simulink library "MCHP_Blockset"  (R2014b)
settings: Solver=ode45  SolverMode=SingleTasking  StartTime=0.0  StopTime=10.0  RelTol=1e-3
InitFcn:
  | disp('MCHP_Blockset_Library_InitFunction');
undefined symbols (not defined in the file): A0, A2, AD0, AVdd, B1, B5, B9, C10, C2, CMP2A, CMP3A, CMP4A, EXTREF1, EXTREF2, gcbh, MaxPer, MCHP_ACC_SAMx_Callback, MCHP_ADC_Callback, MCHP_ADC_HighSpeed_SAR_Callback, MCHP_ADC_HighSpeed_SAR_dsPIC_Callback, MCHP_ADC_SAME5x_Callback, MCHP_AFEC_SAM7x_Callback, MCHP_BUS_I2C_MASTER_callback, MCHP_BUS_SPI_callback, MCHP_C_function_Call_callback, MCHP_CN_Callback, MCHP_COMPARATOR1_callback, MCHP_CompilerOptimisation_Callback, MCHP_DACC_SAMx_Callback, MCHP_Digital_Input_Callback, MCHP_Digital_Output_Read_Callback, MCHP_Digital_Output_Write_Callback, MCHP_Fun, MCHP_HighSpeed_AnalogComparator_Callback, MCHP_IC_Callback, MCHP_IdleTask_Callback, MCHP_Interrupt_Callback, MCHP_Master_Callback, MCHP_MCPWM_Callback, MCHP_MCU_LOAD_Callback, MCHP_MCU_OVERLOAD_Callback, MCHP_MSI_Callback, MCHP_OC_HW_Callback, MCHP_OC_SW_Callback, MCHP_OP_AMP_Callback, MCHP_OrderInOut, MCHP_PDEC_Callback, MCHP_PGA_Callback, MCHP_PWM_Callback, MCHP_PWM_HighSpeed_Override_Callback, MCHP_PWM_HS_FEP_Callback, MCHP_PWM_SAM7x_Callback, MCHP_PWM_SAM7x_Override_Callback, MCHP_QDEC_SAMx_Callback, MCHP_QEI_Callback, MCHP_Scheduler_Options_Callback, MCHP_SECONDARY_CORE_Callback, MCHP_Tasks_State_Callback, MCHP_TCC_PWM_Callback, MCHP_TIMER_Config_Callback ... (+18)
libraries: MCHP_Blockset x2
(part 5 of 9)

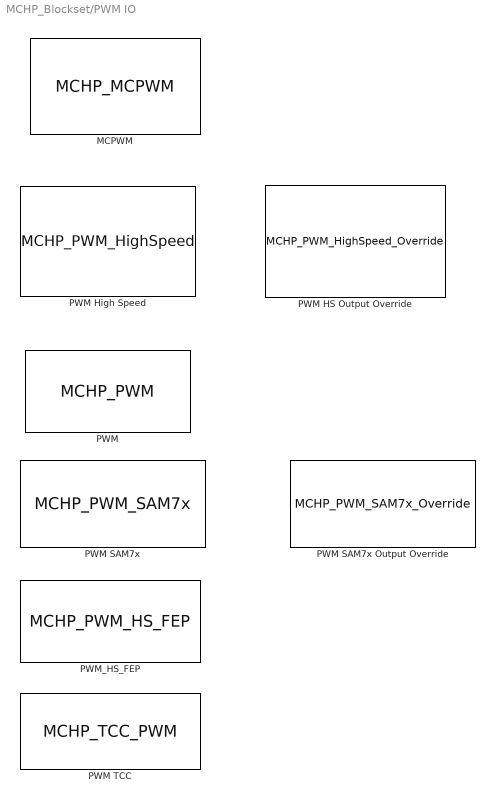
== system MCHP_Blockset/PWM IO ==
  MCPWM : S-Function  Priority=-2000  LoadFcn=MCHP_Fun.Load_EvalIn_ws(gcbh);  InitFcn=MCHP_MCPWM_Callback(gcbh,'InitFcn');  FunctionName=MCHP_MCPWM  Parameters=MCHP_MCPWM_Callback(gcbh,'S_INPUT'),MCHP_MCPWM_Callback(gcbh,'S_OUTPUT'),MCHP_MCPWM_Callback(gcbh,'S_INPUT_Size'),MCHP_MCPWM_Callback(gcbh,'S_OUTPUT_Size'),MCHP_MCPWM_Callback(gcbh,'S_ListCustomDatatype'),SampleTime,0  EnableBusSupport=off  mask(MCPWM PIC32 EF family){PWMx_ECAM_ITB=Common - Edge aligned, PWMx_MTBS=Primary master timer, PWM_ClockResolution=Dynamic Options, PWM_ClockResolution_TXT=auto, MaxPeriod_s=50e-6, InitPeriode_s=50e-6, InitDutyCycleP_s=20e-6, InitDutyCycleS_s=10e-6, InitPhase_s=-1, SampleTime=-1, S_INPUT=[-1], S_INPUT_Size=[3], S_OUTPUT=[], S_OUTPUT_Size=[], S_ListCustomDatatype=S.S_ListCustomDatatype={};, MCHP_USER_INTERRUPTS=0, evalin_ws='', MCHP_PORT={PWMH1 }{PWMH1}32:4:B14;{PWMH2 }{PWMH2}32:4:B12;{PWMH3 }{PWMH3}32:4:B10;{PWML1}{PWML1}32:4:B15;{PWML2}{PWML2}32:4:B13;{PWML3}{PWML3}32:4:B11;, MCHP_MASTERLINK=Export_To_Lib/Microchip Master, MCHP_CRC=1635607, INFO=, PWMx_PMOD=Complementary, PWM1_HL=PWMxH & PWMxL output enabled, PWM1_swap=off, PWM1H_pol=off, PWM1L_pol=off, PWM2_HL=PWMxH & PWMxL output enabled, PWM2_swap=off, PWM2H_pol=off, PWM2L_pol=off, PWM3_HL=PWMxH & PWMxL output enabled, PWM3_swap=off, PWM3H_pol=off, PWM3L_pol=off, PWM4_HL=not used, PWM4_swap=off, PWM4H_pol=off, PWM4L_pol=off, PWM5_HL=not used, PWM5_swap=off, PWM5H_pol=off, PWM5L_pol=off, PWM6_HL=not used, PWM6_swap=off, PWM6H_pol=off, PWM6L_pol=off, PWM7_HL=not used, PWM7_swap=off, PWM7H_pol=off, PWM7L_pol=off, PWM8_HL=not used, PWM8_swap=off, PWM8H_pol=off, PWM8L_pol=off, PWM9_HL=not used, PWM9_swap=off, PWM9H_pol=off, PWM9L_pol=off, PWM10_HL=not used, PWM10_swap=off, PWM10H_pol=off, PWM10L_pol=off, PWM11_HL=not used, PWM11_swap=off, PWM11H_pol=off, PWM11L_pol=off, PWM12_HL=not used, PWM12_swap=off, PWM12H_pol=off, PWM12L_pol=off, Init_SEVTCMP_SSEVTCMP=-1, Init_TRIGx_STRIGx_1=[-1 -1], Init_TRIGx_STRIGx_2=[-1 -1], Init_TRIGx_STRIGx_3=[-1 -1], Init_TRIGx_STRIGx_4=[-1 -1], Init_TRIGx_STRIGx_5=[-1 -1], Init_TRIGx_STRIGx_6=[-1 -1], Init_TRIGx_STRIGx_7=[-1 -1], Init_TRIGx_STRIGx_8=[-1 -1], Init_TRIGx_STRIGx_9=[-1 -1], Init_TRIGx_STRIGx_10=[-1 -1], Init_TRIGx_STRIGx_11=[-1 -1], Init_TRIGx_STRIGx_12=[-1 -1], TRIG_DualTriggerMode=Primary Trigger to ADC is independant, BlockInput_VectorScalar=Vectors (grouped by function), BlockInput_Period=Not a block input, BlockInput_DutyCycle=a Floating Point input within range [0 1], BlockInput_PhaseShift=Not a block input, BlockInput_SEVTCMP=Not a block input, BlockInput_TRIGx=Not a block input, BlockInput_DeadTime=Not a block input, BlockOutput_FaultDisabled=off, BlockOutput_Fault=on, DTC=Disabled, FLTSRC1_DTCMP=Dynamic Options, FLTSRC1_DTCMP_TXT=FLT6 / E13 / Pin[42]  -  Active HIGH, FLTSRC2_DTCMP=Dynamic Options, FLTSRC2_DTCMP_TXT=FLT6 / E13 / Pin[42]  -  Active LOW, FLTSRC3_DTCMP=Dynamic Options, FLTSRC3_DTCMP_TXT=FLT8 / E15 / Pin[44]  -  Active LOW, FLTSRC4_DTCMP=Dynamic Options, FLTSRC4_DTCMP_TXT=FLT3 / C2 / Pin[34]  -  Active HIGH, FLTSRC5_DTCMP=Dynamic Options, FLTSRC5_DTCMP_TXT=FLT3 / C2 / Pin[34]  -  Active HIGH, FLTSRC6_DTCMP=Dynamic Options, FLTSRC6_DTCMP_TXT=FLT3 / C2 / Pin[34]  -  Active HIGH, FLTSRC7_DTCMP=Dynamic Options, FLTSRC7_DTCMP_TXT=FLT3 / C2 / Pin[34]  -  Active HIGH, FLTSRC8_DTCMP=Dynamic Options, FLTSRC8_DTCMP_TXT=FLT3 / C2 / Pin[34]  -  Active HIGH, FLTSRC9_DTCMP=Dynamic Options, FLTSRC9_DTCMP_TXT=FLT3 / C2 / Pin[34]  -  Active HIGH, FLTSRC10_DTCMP=Dynamic Options, FLTSRC10_DTCMP_TXT=FLT3 / C2 / Pin[34]  -  Active HIGH, FLTSRC11_DTCMP=Dynamic Options, FLTSRC11_DTCMP_TXT=FLT3 / C2 / Pin[34]  -  Active HIGH, FLTSRC12_DTCMP=Dynamic Options, FLTSRC12_DTCMP_TXT=FLT3 / C2 / Pin[34]  -  Active HIGH, DeadTime_s=2e-6, DeadTimeAlt_s=2e-6, DeadTimeComp_s=0, FLTMODx=Disabled, FLTSRCx=Dynamic Options, FLTSRCx_TXT=FLT3 / C2 / Pin[34]  -  Active HIGH, FLTDATx=PWM H/L -> 11, CLMODx=Disabled, CLSRCx=Dynamic Options, CLSRCx_TXT=FLT8 / E15 / Pin[44]  -  Active LOW, CLDATx=PWM H/L -> 00, FLTLEBENx=off, CLLEBENx=off, LeadEdgeBlkPer_s=5e-7, PHRx=off, PHFx=off, PLRx=off, PLFx=off}
      mask prompts: PWMx_ECAM_ITB "Period :"; PWMx_MTBS "Clock source :"; PWM_ClockResolution "Clock source resolution : [PWM res 8.333(ns) => periode up to 546(us) ]"; PWM_ClockResolution_TXT "<empty>"; MaxPeriod_s "Max Period (s) : PWM1max=PWM2max=PWM3max=6000 (12.55bits width)  represent 50(us)"; InitPeriode_s "Initial Period (s) :"; InitDutyCycleP_s "Initial Duty Cycle (s)"; InitDutyCycleS_s "Initial second half Duty Cycle (s)"; InitPhase_s "Initial Phase (s) :"; SampleTime "Block output sample time"; INFO "Infos"; PWMx_PMOD "High/Low side Mode :"; PWM1_HL "PWM 1 Channel"; PWM1_swap "Swap PWM1_H and PWM1_L"; PWM1H_pol "invert PWM1_H output polarity ( B14 [4] active low )"; PWM1L_pol "invert PWM1_L output polarity ( B15 [5] active low )"; PWM2_HL "PWM 2 Channel"; PWM2_swap "Swap PWM2_H and PWM2_L"; PWM2H_pol "invert PWM2_H output polarity ( B12 [98] active low )"; PWM2L_pol "invert PWM2_L output polarity ( B13 [99] active low )"; PWM3_HL "PWM 3 Channel"; PWM3_swap "Swap PWM3_H and PWM3_L"; PWM3H_pol "invert PWM3_H output polarity ( B10 [93] active low )"; PWM3L_pol "invert PWM3_L output polarity ( B11 [94] active low )"; PWM4_HL "PWM 4 Channel"; PWM4_swap "Swap PWM4_H and PWM4_L"; PWM4H_pol "invert PWM4_H output polarity ( A10 [100] active low )"; PWM4L_pol "invert PWM4_L output polarity ( A7 [3] active low )"; PWM5_HL "PWM 5 Channel"; PWM5_swap "Swap PWM5_H and PWM5_L"; PWM5H_pol "invert PWM5_H output polarity ( D2 [7] active low )"; PWM5L_pol "invert PWM5_L output polarity ( D1 [6] active low )"; PWM6_HL "PWM 6 Channel"; PWM6_swap "Swap PWM6_H and PWM6_L"; PWM6H_pol "invert PWM6_H output polarity ( D4 [9] active low )"; PWM6L_pol "invert PWM6_L output polarity ( D3 [8] active low )"; PWM7_HL "PWM 7 Channel"; PWM7_swap "Swap PWM7_H and PWM7_L"; PWM7H_pol "invert PWM7_H output polarity ( B15 [5] active low )"; PWM7L_pol "<empty>"; PWM8_HL "PWM 8 Channel"; PWM8_swap "Swap PWM8_H and PWM8_L"; PWM8H_pol "invert PWM8_H output polarity ( B13 [99] active low )"; PWM8L_pol "<empty>"; PWM9_HL "PWM 9 Channel"; PWM9_swap "Swap PWM9_H and PWM9_L"; PWM9H_pol "invert PWM9_H output polarity ( B11 [94] active low )"; PWM9L_pol "<empty>"; PWM10_HL "PWM 10 Channel"; PWM10_swap "Swap PWM10_H and PWM10_L"; PWM10H_pol "invert PWM10_H output polarity ( A7 [3] active low )"; PWM10L_pol "<empty>"; PWM11_HL "PWM 11 Channel"; PWM11_swap "Swap PWM11_H and PWM11_L"; PWM11H_pol "invert PWM11_H output polarity ( F0 [87] active low )"; PWM11L_pol "invert PWM11_L output polarity ( F1 [88] active low )"; PWM12_HL "PWM 12 Channel"; PWM12_swap "Swap PWM12_H and PWM12_L"; PWM12H_pol "invert PWM12_H output polarity ( D5 [82] active low )"; PWM12L_pol "invert PWM12_L output polarity ( D6 [83] active low )"; Init_SEVTCMP_SSEVTCMP "Master time base trigger initial value (s)"; Init_TRIGx_STRIGx_1 "PWM1 [Primary Secondary] Trigger initial value (s)"; Init_TRIGx_STRIGx_2 "PWM2 [Primary Secondary] Trigger initial value (s)"; Init_TRIGx_STRIGx_3 "PWM3 [Primary Secondary] Trigger initial value (s)"; Init_TRIGx_STRIGx_4 "PWM4 [Primary Secondary] Trigger initial value (s)"; Init_TRIGx_STRIGx_5 "PWM5 [Primary Secondary] Trigger initial value (s)"; Init_TRIGx_STRIGx_6 "PWM6 [Primary Secondary] Trigger initial value (s)"; Init_TRIGx_STRIGx_7 "PWM7 [Primary Secondary] Trigger initial value (s)"; Init_TRIGx_STRIGx_8 "PWM8 [Primary Secondary] Trigger initial value (s)"; Init_TRIGx_STRIGx_9 "PWM9 [Primary Secondary] Trigger initial value (s)"; Init_TRIGx_STRIGx_10 "PWM10 [Primary Secondary] Trigger initial value (s)"; Init_TRIGx_STRIGx_11 "PWM11 [Primary Secondary] Trigger initial value (s)"; Init_TRIGx_STRIGx_12 "PWM12 [Primary Secondary] Trigger initial value (s)"; TRIG_DualTriggerMode "Primary trigger to ADC"; BlockInput_VectorScalar "Block input format:"; BlockInput_Period "Period :"; BlockInput_DutyCycle "Duty Cycle :"; BlockInput_PhaseShift "Phase Shift :"; BlockInput_SEVTCMP "Master Time base event trigger :"; BlockInput_TRIGx "PWM Channel Primary/Secondary trigger :"; BlockInput_DeadTime "Dead Time :"; BlockOutput_FaultDisabled "PWM Fault State is a block Output"; BlockOutput_Fault "PWM Fault State is a block Output"; DTC "+++ Dead Time : +++"; FLTSRC1_DTCMP "Fault input pin for PWM 1"; FLTSRC1_DTCMP_TXT "<empty>"; FLTSRC2_DTCMP "Fault input pin for PWM 2"; FLTSRC2_DTCMP_TXT "<empty>"; FLTSRC3_DTCMP "Fault input pin for PWM 3"; FLTSRC3_DTCMP_TXT "<empty>"; FLTSRC4_DTCMP "Fault input pin for PWM 4"; FLTSRC4_DTCMP_TXT "<empty>"; FLTSRC5_DTCMP "Fault input pin for PWM 5"; FLTSRC5_DTCMP_TXT "<empty>"; FLTSRC6_DTCMP "Fault input pin for PWM 6"; FLTSRC6_DTCMP_TXT "<empty>"; FLTSRC7_DTCMP "Fault input pin for PWM 7"; FLTSRC7_DTCMP_TXT "<empty>"; FLTSRC8_DTCMP "Fault input pin for PWM 8"; FLTSRC8_DTCMP_TXT "<empty>"; FLTSRC9_DTCMP "Fault input pin for PWM 9"; FLTSRC9_DTCMP_TXT "<empty>"; FLTSRC10_DTCMP "Fault input pin for PWM 10"; FLTSRC10_DTCMP_TXT "<empty>"; FLTSRC11_DTCMP "Fault input pin for PWM 11"; FLTSRC11_DTCMP_TXT "<empty>"; FLTSRC12_DTCMP "Fault input pin for PWM 12"; FLTSRC12_DTCMP_TXT "<empty>"; DeadTime_s "Positive dead time on rising edge of PWM_H (s) - (DTRx)"; DeadTimeAlt_s "Positive dead time on rising edge of PWM_L (s) - (ALTDTRx)"; DeadTimeComp_s "Dead Time Compensation value"; FLTMODx "+++ Fault protection : +++"; FLTSRCx "Fault protection input pin"; FLTSRCx_TXT "<empty>"; FLTDATx "Failt protection safe state :"; CLMODx "+++ Current Limit : +++"; CLSRCx "Current-Limit input pin"; CLSRCx_TXT "<empty>"; CLDATx "Current limit safe state :"; FLTLEBENx "Enable Leading-Edge Blanking to remove glitch on Fault input"; CLLEBENx "Enable Leading-Edge Blanking to remove glitch on Current-Limit input"; LeadEdgeBlkPer_s "Blanking period (s) :"; PHRx "Rising edge of PWM_H trig Leading-Edge Blanking"; PHFx "Falling edge of PWM_H trig Leading-Edge Blanking"; PLRx "Rising edge of PWM_L trig Leading-Edge Blanking"; PLFx "Falling edge of PWM_L trig Leading-Edge Blanking"
      mask help:
      | Multiple instance of this MCPWM block might be used within a model to
      |   + set PWM channels with differents characteristics
      |   + update block input at differents time or on specific conditions
      | Model will not compiled if several MCPWM settings does not comply with hardware capabilities
      |
      | Initial values fields tips (when applicable)
      |   + Scalar input set the same value for all channels enabled.
      |   + Vector  set values for respective channels enabled (first value, first enabled channel...)
      |   + -1 means not used. (for scalar or vector representation)
      mask init:
      | MCHP_MCPWM_Callback(gcbh,'INITIALISATION');
      settings: CopyFcn=MCHP_MCPWM_Callback(gcbh,'CopyFcn');  PreSaveFcn=MCHP_Fun.PreSaveFcn_DynamicOptions(gcbh);  OpenFcn=MCHP_MCPWM_Callback(gcbh,'OPEN');
      mask TypeOptions PWMx_ECAM_ITB: Common - Edge aligned | Common - Center aligned - Symetric | Common - Center aligned - Symetric - Enhanced resolution | Common - Center aligned - Asymetric with double update | Common - Center aligned - Asymetric with simultaneous update | --- | Independant - Edge aligned | Independant - Center aligned - Symetric | Independant - Center aligned - Symetric - Enhanced resolution | Independant - Center aligned - Asymetric with double update | Independant - Center aligned - Asymetric with simultaneous update
      mask Callback PWMx_ECAM_ITB: MCHP_MCPWM_Callback(gcbh,'UpdateGUI');
      mask TypeOptions PWMx_MTBS: Primary master timer | Secondary master timer
      mask TypeOptions PWM_ClockResolution: Dynamic Options
      mask TypeOptions PWMx_PMOD: Complementary | Redundant | Push Pull
      mask TypeOptions PWM1_HL: PWMxH & PWMxL output enabled | PWMxH output enabled | PWMxL output enabled | not used | Enabled with NO output
      mask Callback PWM1_HL: MCHP_MCPWM_Callback(gcbh,'UpdateGUI');
      mask TypeOptions PWM2_HL: PWMxH & PWMxL output enabled | PWMxH output enabled | PWMxL output enabled | not used | Enabled with NO output
      mask Callback PWM2_HL: MCHP_MCPWM_Callback(gcbh,'UpdateGUI');
      mask TypeOptions PWM3_HL: PWMxH & PWMxL output enabled | PWMxH output enabled | PWMxL output enabled | not used | Enabled with NO output
      mask Callback PWM3_HL: MCHP_MCPWM_Callback(gcbh,'UpdateGUI');
      mask TypeOptions PWM4_HL: PWMxH & PWMxL output enabled | PWMxH output enabled | PWMxL output enabled | not used | Enabled with NO output
      mask Callback PWM4_HL: MCHP_MCPWM_Callback(gcbh,'UpdateGUI');
      mask TypeOptions PWM5_HL: PWMxH & PWMxL output enabled | PWMxH output enabled | PWMxL output enabled | not used | Enabled with NO output
      mask Callback PWM5_HL: MCHP_MCPWM_Callback(gcbh,'UpdateGUI');
      mask TypeOptions PWM6_HL: PWMxH & PWMxL output enabled | PWMxH output enabled | PWMxL output enabled | not used | Enabled with NO output
      mask Callback PWM6_HL: MCHP_MCPWM_Callback(gcbh,'UpdateGUI');
      mask TypeOptions PWM7_HL: PWMxH & PWMxL output enabled | PWMxH output enabled | PWMxL output enabled | not used | Enabled with NO output
      mask Callback PWM7_HL: MCHP_MCPWM_Callback(gcbh,'UpdateGUI');
      mask TypeOptions PWM8_HL: PWMxH & PWMxL output enabled | PWMxH output enabled | PWMxL output enabled | not used | Enabled with NO output
      mask Callback PWM8_HL: MCHP_MCPWM_Callback(gcbh,'UpdateGUI');
      mask TypeOptions PWM9_HL: PWMxH & PWMxL output enabled | PWMxH output enabled | PWMxL output enabled | not used | Enabled with NO output
      mask Callback PWM9_HL: MCHP_MCPWM_Callback(gcbh,'UpdateGUI');
      mask TypeOptions PWM10_HL: PWMxH & PWMxL output enabled | PWMxH output enabled | PWMxL output enabled | not used | Enabled with NO output
      mask Callback PWM10_HL: MCHP_MCPWM_Callback(gcbh,'UpdateGUI');
      mask TypeOptions PWM11_HL: PWMxH & PWMxL output enabled | PWMxH output enabled | PWMxL output enabled | not used | Enabled with NO output
      mask Callback PWM11_HL: MCHP_MCPWM_Callback(gcbh,'UpdateGUI');
      mask TypeOptions PWM12_HL: PWMxH & PWMxL output enabled | PWMxH output enabled | PWMxL output enabled | not used | Enabled with NO output
      mask Callback PWM12_HL: MCHP_MCPWM_Callback(gcbh,'UpdateGUI');
      mask TypeOptions TRIG_DualTriggerMode: Primary Trigger to ADC is independant | Primary trigger to ADC merge Primary and Secondary trigger pulse
      mask TypeOptions BlockInput_VectorScalar: Independant Scalar | Vectors (grouped by function)
      mask TypeOptions BlockInput_Period: Not a block input | a Uint raw input (PWMxmax variable represent max period) | a Floating Point input within range [0 1]  | a Floating Point input within range [-1 1] | a Floating Point input with physical scaling in (s)
      mask TypeOptions BlockInput_DutyCycle: Not a block input | a Uint raw input (PWMxmax variable represent max period) | a Floating Point input within range [0 1]  | a Floating Point input within range [-1 1] | a Floating Point input with physical scaling in (s)
      mask TypeOptions BlockInput_PhaseShift: Not a block input | a Uint raw input (PWMxmax variable represent max period) | a Floating Point input within range [0 1]  | a Floating Point input within range [-1 1] | a Floating Point input with physical scaling in (s)
      mask TypeOptions BlockInput_SEVTCMP: Not a block input | a Uint raw input (PWMxmax variable represent max period) | a Floating Point input within range [0 1]  | a Floating Point input within range [-1 1] | a Floating Point input with physical scaling in (s)
      mask TypeOptions BlockInput_TRIGx: Not a block input | a Uint raw input (PWMxmax variable represent max period) | a Floating Point input within range [0 1]  | a Floating Point input within range [-1 1] | a Floating Point input with physical scaling in (s)
      mask TypeOptions BlockInput_DeadTime: Not a block input | a Uint raw input (PWMxmax variable represent max period) | a Floating Point input within range [0 1]  | a Floating Point input within range [-1 1] | a Floating Point input with physical scaling in (s)
      mask TypeOptions DTC: Disabled | Positive dead time (ensure period of time with PWM_H and PWM_L disasserted) | Negative dead time (edge aligned only) | Positive dead time with compensation mode
      mask Callback DTC: MCHP_MCPWM_Callback(gcbh,'UpdateGUI');
      mask TypeOptions FLTSRC1_DTCMP: Dynamic Options
      mask TypeOptions FLTSRC2_DTCMP: Dynamic Options
      mask TypeOptions FLTSRC3_DTCMP: Dynamic Options
      mask TypeOptions FLTSRC4_DTCMP: Dynamic Options
      mask TypeOptions FLTSRC5_DTCMP: Dynamic Options
      mask TypeOptions FLTSRC6_DTCMP: Dynamic Options
      mask TypeOptions FLTSRC7_DTCMP: Dynamic Options
      mask TypeOptions FLTSRC8_DTCMP: Dynamic Options
      mask TypeOptions FLTSRC9_DTCMP: Dynamic Options
      mask TypeOptions FLTSRC10_DTCMP: Dynamic Options
      mask TypeOptions FLTSRC11_DTCMP: Dynamic Options
      mask TypeOptions FLTSRC12_DTCMP: Dynamic Options
      mask TypeOptions FLTMODx: Disabled | Force PWM output for current cycle. Enable PWM on next cycle | Force PWM output until the FLT block input is 1
      mask Callback FLTMODx: MCHP_MCPWM_Callback(gcbh,'UpdateGUI');
      mask TypeOptions FLTSRCx: Dynamic Options
      mask TypeOptions FLTDATx: PWM H/L -> 00 | PWM H/L -> 01 | PWM H/L -> 10 | PWM H/L -> 11 | Not forced
      mask TypeOptions CLMODx: Disabled | Enabled
      mask Callback CLMODx: MCHP_MCPWM_Callback(gcbh,'UpdateGUI');
      mask TypeOptions CLSRCx: Dynamic Options
      mask TypeOptions CLDATx: PWM H/L -> 00 | PWM H/L -> 01 | PWM H/L -> 10 | PWM H/L -> 11 | Not forced
      mask Callback FLTLEBENx: MCHP_MCPWM_Callback(gcbh,'UpdateGUI');
      mask Callback CLLEBENx: MCHP_MCPWM_Callback(gcbh,'UpdateGUI');
      mask Display:
      | fprintf('          PWM\n\n          PIC32 EF');
      | port_label('input',1,'DutyCycle[1 2 3]');
  PWM : S-Function  LoadFcn=MCHP_Fun.Load_EvalIn_ws(gcbh);  InitFcn=MCHP_PWM_Callback(gcbh,'InitFcn');  FunctionName=MCHP_PWM  Parameters=SampleTime,MCHP_PWM_Callback(gcbh,'S_INPUT'),MCHP_PWM_Callback(gcbh,'S_OUTPUT'),0  EnableBusSupport=off  mask(PWM Motor Output){PWM_REF=1, ChannelHighLowChk=off, Channel=[1  3], ChannelHigh=[1 2 4], InitialPeriod=.001, InputPeriodeChk=off, CAM=on, IUE=on, evalin_ws='', Info=PWM1max = 39997  ;   % ==>  15.2876 bits, MCHP_MASTERLINK=dsPICDEM_MCLV_V1_33FJ256MC710A/Microchip Master, MCHP_PORT={PWM Fault}{FLTA}5:0:E8;, ADC_VARTRIG={PWM Primary Special Event Trigger;6}, SampleTime=-1, DeadTimePrescaleA=.005*1e-3, DeadTimePrescaleB=.010*1e-3, DTPWM1a=Prescaler A, DTPWM1i=Prescaler B, DTPWM2a=Prescaler A, DTPWM2i=Prescaler A, DTPWM3a=Prescaler A, DTPWM3i=Prescaler A, DTPWM4a=Prescaler A, DTPWM4i=Prescaler A, PIN_FaultA=Dynamic Options, PIN_FaultA_TXT=Dynamic Options, FAULTA_FLATM=Re-Enable PWM when Fault Pin is desactivated, FaultA_Output=off, FaultA_PWM1_State=H/L ==> 00, FaultA_PWM2_State=H/L ==> 00, FaultA_PWM3_State=H/L ==> 00, FaultA_PWM4_State=No Changes (PWM), PIN_FaultB=Dynamic Options, PIN_FaultB_TXT=Dynamic Options, FAULTB_FLBTM=Re-Enable PWM when Fault Pin is desactivated, FaultB_Output=off, FaultB_PWM1_State=No Changes (PWM), FaultB_PWM2_State=No Changes (PWM), FaultB_PWM3_State=No Changes (PWM), FaultB_PWM4_State=No Changes (PWM), PxSECMP=.0005, PxSECMPBlkInChk=off, OVDCONChk=off, Parameter43=0}
      mask prompts: PWM_REF "PWM"; ChannelHighLowChk "Distinct Enable of PWM High and PWM Low channels"; Channel "Output Channels (High and Low) : [1  2  3  4]"; ChannelHigh "Output Channels (High) : [1  2  3  4]"; InitialPeriod "Periode (s)"; InputPeriodeChk "Input Periode (otherwise set to  max periode)"; CAM "Center Aligned Mode"; IUE "Immediate Update"; DeadTimePrescaleA "Dead Time A: 5e-06s    Max is 1.26e-05s"; DeadTimePrescaleB "Dead Time B: 1e-05s    Max is 1.26e-05s"; DTPWM1a "Dead Time PWM1 Active"; DTPWM1i "Dead Time PWM1 Inactive"; DTPWM2a "Dead Time PWM2 Active"; DTPWM2i "Dead Time PWM2 Inactive"; DTPWM3a "Dead Time PWM3 Active"; DTPWM3i "Dead Time PWM3 Inactive"; DTPWM4a "Dead Time PWM4 Active"; DTPWM4i "Dead Time PWM4 Inactive"; PIN_FaultA "Fault A Pin"; FAULTA_FLATM "Fault A behaviour"; FaultA_Output "Fault A Detection block output"; FaultA_PWM1_State "Fault  A: PWM1 H/L  Pins State :"; FaultA_PWM2_State "Fault  A: PWM2 H/L  Pins State :"; FaultA_PWM3_State "Fault  A: PWM3 H/L  Pins State :"; FaultA_PWM4_State "Fault  A: PWM4 H/L  Pins State :"; PIN_FaultB "Fault B Pin"; FAULTB_FLBTM "Fault B behaviour"; FaultB_Output "Fault B Detection block output"; FaultB_PWM1_State "Fault  B: PWM1 H/L  Pins State :"; FaultB_PWM2_State "Fault  B: PWM2 H/L  Pins State :"; FaultB_PWM3_State "Fault  B: PWM3 H/L  Pins State :"; FaultB_PWM4_State "Fault  B: PWM4 H/L  Pins State :"; PxSECMP "Special Event Trigger (s)"; PxSECMPBlkInChk "Special Event Trigger is a block input"; OVDCONChk "Override register input (OVDCON)"
      mask help:
      | floor(PWM[x]max/2) value is the max value period input.
      | PWM[x]max value is the max value for Duty Cycle.
      | Theses max values correspond to the max period time set within the block.
      mask init:
      | MCHP_PWM_Callback(gcbh,'INITIALISATION');
      settings: CopyFcn=MCHP_PWM_Callback(gcbh,'InitFcn');  PreSaveFcn=MCHP_Fun.PreSaveFcn_DynamicOptions(gcbh);  OpenFcn=MCHP_PWM_Callback(gcbh,'OPEN');
      mask TypeOptions PWM_REF: 1 | 2 | Duplicate ports for PWM 1 | Duplicate ports for PWM 2
      mask Callback ChannelHighLowChk: MCHP_PWM_Callback(gcbh,'ChannelHighLowChk');
      mask TypeOptions DTPWM1a: Prescaler A | Prescaler B
      mask TypeOptions DTPWM1i: Prescaler A | Prescaler B
      mask TypeOptions DTPWM2a: Prescaler A | Prescaler B
      mask TypeOptions DTPWM2i: Prescaler A | Prescaler B
      mask TypeOptions DTPWM3a: Prescaler A | Prescaler B
      mask TypeOptions DTPWM3i: Prescaler A | Prescaler B
      mask TypeOptions DTPWM4a: Prescaler A | Prescaler B
      mask TypeOptions DTPWM4i: Prescaler A | Prescaler B
      mask TypeOptions PIN_FaultA: Dynamic Options
      mask Callback PIN_FaultA: MCHP_Fun.BlockUpdate(gcbh);
      mask TypeOptions FAULTA_FLATM: Re-Enable PWM when Fault Pin is desactivated | Use Re-Enable block input after Fault is detected
      mask TypeOptions FaultA_PWM1_State: No Changes (PWM) | H/L ==> 00 | H/L ==> 01 | H/L ==> 10 | H/L ==> 11
      mask TypeOptions FaultA_PWM2_State: No Changes (PWM) | H/L ==> 00 | H/L ==> 01 | H/L ==> 10 | H/L ==> 11
      mask TypeOptions FaultA_PWM3_State: No Changes (PWM) | H/L ==> 00 | H/L ==> 01 | H/L ==> 10 | H/L ==> 11
      mask TypeOptions FaultA_PWM4_State: No Changes (PWM) | H/L ==> 00 | H/L ==> 01 | H/L ==> 10 | H/L ==> 11
      mask TypeOptions PIN_FaultB: Dynamic Options
      mask Callback PIN_FaultB: MCHP_Fun.BlockUpdate(gcbh);
      mask TypeOptions FAULTB_FLBTM: Re-Enable PWM when Fault Pin is desactivated | Use Re-Enable block input after Fault is detected
      mask TypeOptions FaultB_PWM1_State: No Changes (PWM) | H/L ==> 00 | H/L ==> 01 | H/L ==> 10 | H/L ==> 11
      mask TypeOptions FaultB_PWM2_State: No Changes (PWM) | H/L ==> 00 | H/L ==> 01 | H/L ==> 10 | H/L ==> 11
      mask TypeOptions FaultB_PWM3_State: No Changes (PWM) | H/L ==> 00 | H/L ==> 01 | H/L ==> 10 | H/L ==> 11
      mask TypeOptions FaultB_PWM4_State: No Changes (PWM) | H/L ==> 00 | H/L ==> 01 | H/L ==> 10 | H/L ==> 11
      mask Display:
      | MCHP_DrawLogo;
      | fprintf('PWM ');
  PWM HS Output Override : S-Function  InitFcn=MCHP_PWM_HighSpeed_Override_Callback(gcbh,'InitFcn');  FunctionName=MCHP_PWM_HighSpeed_Override  Parameters=MCHP_PWM_HighSpeed_Override_Callback(gcb,'S_INPUT'),MCHP_PWM_HighSpeed_Override_Callback(gcb,'S_OUTPUT'),MCHP_PWM_HighSpeed_Override_Callback(gcb,'S_INPUT_Size'),MCHP_PWM_HighSpeed_Override_Callback(gcb,'S_OUTPUT_Size'),[],SampleTime,0  EnableBusSupport=off  mask(High Speed PWM Override outputs){PWM_Refs=[1 2  3], OVEREN_OVERDAT_Initial=[0 1 15], MCHP_MASTERLINK=UTB_33EP512MU810_PWM_HS_Override/Microchip Master, S_INPUT=[5  5  5], S_INPUT_Size=[1  1  1], S_OUTPUT=[], S_OUTPUT_Size=[], SampleTime=-1}
      mask prompts: PWM_Refs "PWM Channel Reference to Override within [1 - 6]"; OVEREN_OVERDAT_Initial "Initial Values"; SampleTime "Sample Time"
      mask help:
      | A block PWM HS must be present to use the PWM High Speed Peripheral.
      |
      | This block allows to force PWM output.
      | Block inputs and Dialog Initial value have the following coding scheme:
      | bit 3: value 1 override the PWMxH pin with bit 1 value; value 0 provide PWM generator output
      | bit 2: value 1 override the PWMxL pin with bit 0 value; value 0 provide PWM generator output
      | bit 1: PWMxH override data
      | bit 0: PWMxH override data
      mask init:
      | MCHP_PWM_HighSpeed_Override_Callback(gcbh,'INITIALISATION');
      settings: CopyFcn=MCHP_PWM_HighSpeed_Override_Callback(gcbh,'CopyFcn');  PreSaveFcn=MCHP_Fun.PreSaveFcn_DynamicOptions(gcbh);  OpenFcn=MCHP_PWM_HighSpeed_Override_Callback(gcbh,'OPEN');
      mask Callback S_INPUT_Size: MCHP_Fun.BlockUpdate(gcbh);
      mask Display:
      | MCHP_DrawLogo;disp('High Speed\nPWM Output Override')
      | port_label('input',1,'OvDr 1');
      | port_label('input',2,'OvDr 2');
      | port_label('input',3,'OvDr 3');
  PWM High Speed : S-Function  LoadFcn=MCHP_Fun.Load_EvalIn_ws(gcbh);  FunctionName=MCHP_PWM_HighSpeed  Parameters=SampleTime,MCHP_QEI_Callback(gcbh,'S_INPUT'),MCHP_QEI_Callback(gcbh,'S_OUTPUT'),MCHP_QEI_Callback(gcbh,'S_INPUT_Size'),MCHP_QEI_Callback(gcbh,'S_OUTPUT_Size'),S_DWORK_Type,S_DWORK_Size,0  EnableBusSupport=off  mask{pop1=[1], chk1=[1  1  1  0  0], chkHL1=[1  1  1  0  0  1  1 ; 1  1  1  0  0  1  1], maxP1={ '0.001','0.001','0.001','0.001','0.001','0.001','0.001';'0.001','0.001','1e-06','0.001','0.001','0.001','0.001'}, InitP2={ '0.001','0.001','0.001','0.001','0.001','0.001','0.001';'0.001','0.001','0.001','0.001','0.001','0.001','0.001'}, chkP2=[0  0  0  1  1  1  1 ; 1  0  0  1  1  1  1], InitDC={ '10','20','30','0.001','50','50','50';'0.001','0.001','0.001','0.001','0.001','50','50'}, chkDC=[1  1  1  1  1  1  1 ; 0  0  0  1  1  1  1], InitPh={ '0','0','0','0.001','0.001','0.001','0.001';'0','0','0','0.001','0.001','0.001','0.001'}, chkPh=[0  0  0  1  1  1  1 ; 0  0  0  1  1  1  1], edSEvTrigx={ '0.0','-1','-1','-1','-1','-1','-1'}, chkSEvTrigx=[0  0  0  1  1  1  1], popFlt=[1  1  1  1  1  1  1], popFltPin=[30  25  24  16  16  16  16], popFltPinRp=[1  1  1  1  1  1  1], popFltActivH=[2  2  1  1  1  1  1], popFltForceH=[2  2  2  2  2  2  2], popFltForceL=[2  1  2  1  1  1  1], chkFltBlkOut=[0  0  0  0  0  0  0], popIndepFaultMode=[1  1  1  1  1  1  1], popCurEnabled=[1  1  1  1  1  1  1], popCurPin=[33  31  32  16  16  16  16], popCurActiveH=[1  1  1  1  1  1  1], popCurForceH=[2  1  2  1  1  1  1], popCurForceL=[2  1  2  1  1  1  1], ChkCurBlkOut=[1  0  0  0  0  0  0], ChkCurBlkOutTime=[1  0  1  0  0  0  0], popBLANKSEL=[1  1  1  1  1  1  1], popBPHHBPHL=[1  1  1  1  1  1  1], popBPLHBPLL=[1  1  1  1  1  1  1], popFLTLEBEN_CLLEBEN=[1  1  1  1  1  1  1], popPHR_PHF=[2  1  1  1  1  1  1], popPLR_PLF=[3  1  1  1  1  1  1], edLEB={ '100e-9','50e-9','150e-9','50e-9','50e-9','50e-9','50e-9'}, popDT=[3  3  3  3  3  3  3], edDTRx={ '0.02','1e-05','0.001','1e-05','1e-05','1e-05','1e-05'}, edAltDTRx={ '1e-05','0.0001','1e-05','1e-05','1e-05','1e-05','1e-05'}, S_INPUT=[5  5  5  5], S_INPUT_Size=[1 1 1 1], S_OUTPUT=[], S_OUTPUT_Size=[], S_DWORK_Type=[], S_DWORK_Size=[], ADC_VARTRIG={PWM Primary Special Event Trigger;6}, evalin_ws='', SampleTime=-1, ORDERING=None, MCHP_PORT={PWM1H}{PWM1H}4:4:A4;{PWM1L}{PWM1L}4:4:A3;{PWM2H}{PWM2H}4:4:B13;{PWM2L}{PWM2L}4:4:B14;{PWM3H}{PWM3H}4:4:B11;{PWM3L}{PWM3L}4:4:B12;, MCHP_MASTERLINK=Export_PWM/Microchip Master, MCHP_VERSION=v3.39, Parameter50=0}
      mask prompts: pop1 "PMOD ITB"; chk1 "MDCS CAM IU"; chkHL1 "PWM Enable"; maxP1 "PWM Max Period"; InitP2 "Initial Period"; chkP2 "Period Checkbox"; InitDC "Initial DutyCycle"; chkDC "DutyCycle Checkbox"; InitPh "Initial Phase"; chkPh "Phase Checkox"; edSEvTrigx "Initial Special Event Trigger"; chkSEvTrigx "Special Event Trigger Checkbox"; popFlt "Fault Enable/Disable mode"; popFltPin "Fault pin"; popFltPinRp "Fault pin Remappable"; popFltActivH "Fault pin Active High/Low"; popFltForceH "Fault Force H pins"; popFltForceL "Fault Force L pins"; chkFltBlkOut "Block Output Fault state"; popIndepFaultMode "Independant Fault"; popCurEnabled "Fault Current Enabled/Disabled"; popCurPin "Current Limit Pin"; popCurActiveH "Current Limit Pin Active"; popCurForceH "Current Limit H pins"; popCurForceL "Current Limit L pins"; ChkCurBlkOut "Block Output Current Limit State"; ChkCurBlkOutTime "Block Output Current Limit Timing"; popDT "Dead Time Enable / disable"; edDTRx "Dead Time"; edAltDTRx "Alternate Dead Time"; SampleTime "Sample Time"; ORDERING "Block execution ordering"
      mask init:
      | MCHP_PWM_HighSpeed_Callback(gcbh,'INITIALISATION');
      settings: DeleteFcn=MCHP_PWM_HighSpeed_gui(gcbh,'DELETE');  ModelCloseFcn=MCHP_PWM_HighSpeed_gui(gcbh,'MODELCLOSE');  OpenFcn=MCHP_PWM_HighSpeed_gui(gcbh,'OPEN');
      mask TypeOptions ORDERING: None | Input | Output | Input & Output
      mask Display:
      | MCHP_DrawLogo;fprintf('High Speed\nPWM');
      | port_label('input',1,'DutyCycle 1');
      | port_label('input',2,'DutyCycle 2');
      | port_label('input',3,'DutyCycle 3');
  PWM SAM7x : S-Function  Priority=-2000  LoadFcn=MCHP_Fun.Load_EvalIn_ws(gcbh);  InitFcn=MCHP_PWM_SAM7x_Callback(gcbh,'InitFcn');  FunctionName=MCHP_PWM_SAM7x  Parameters=MCHP_PWM_SAM7x_Callback(gcbh,'S_INPUT'),MCHP_PWM_SAM7x_Callback(gcbh,'S_OUTPUT'),MCHP_PWM_SAM7x_Callback(gcbh,'S_INPUT_Size'),MCHP_PWM_SAM7x_Callback(gcbh,'S_OUTPUT_Size'),MCHP_PWM_SAM7x_Callback(gcbh,'S_ListCustomDatatype'),SampleTime,0  EnableBusSupport=off  mask(PWM for SAMx7){PWMx=PWM Controller 0, MaxPeriod_s=1e-3, PWM0_pinH0=Dynamic Options, PWM0_pinH0_TXT=PA11 / Pin[64], PWM0_pinL0=Dynamic Options, PWM0_pinL0_TXT=PD24 / Pin[55], PWM0_pinH1=Dynamic Options, PWM0_pinH1_TXT=PA2 / Pin[93], PWM0_pinL1=Dynamic Options, PWM0_pinL1_TXT=PA20 / Pin[22], PWM0_pinH2=Dynamic Options, PWM0_pinH2_TXT=PA13 / Pin[42], PWM0_pinL2=Dynamic Options, PWM0_pinL2_TXT=PA16 / Pin[45], PWM0_pinH3=Dynamic Options, PWM0_pinH3_TXT=Not Used, PWM0_pinL3=Dynamic Options, PWM0_pinL3_TXT=Not Used, PWM1_pinH0=Dynamic Options, PWM1_pinH0_TXT=Not Used, PWM1_pinL0=Dynamic Options, PWM1_pinL0_TXT=Not Used, PWM1_pinH1=Dynamic Options, PWM1_pinH1_TXT=Not Used, PWM1_pinL1=Dynamic Options, PWM1_pinL1_TXT=Not Used, PWM1_pinH2=Dynamic Options, PWM1_pinH2_TXT=Not Used, PWM1_pinL2=Dynamic Options, PWM1_pinL2_TXT=Not Used, PWM1_pinH3=Dynamic Options, PWM1_pinH3_TXT=Not Used, PWM1_pinL3=Dynamic Options, PWM1_pinL3_TXT=Not Used, PWM_Centered=on, PWM_SyncWithPWM0=on, PushPull_Mode=off, SampleTime=-1, S_INPUT=[-1], S_INPUT_Size=[3], S_OUTPUT=[], S_OUTPUT_Size=[], S_ListCustomDatatype=S.S_ListCustomDatatype={};, evalin_ws=PWM0max0=MCHP_Fun.Hex2num('40E24F8000000000');PWM1max0=MCHP_Fun.Hex2num('40E24F8000000000');PWM2max0=MCHP_Fun.Hex2num('40E24F8000000000');, MCHP_PWMC_CLOCK_REQUEST='', MCHP_PWMC_CLOCK_RESULT='', MCHP_USER_INTERRUPTS=0, MCHP_PORT={PWM0H0 }{PWMH0}4:1:P11;{PWM0L0 }{PWML0}4:1:P120;{PWM0H1 }{PWMH1}4:1:P2;{PWM0L1 }{PWML1}4:1:P20;{PWM0H2 }{PWMH2}4:1:P13;{PWM0L2 }{PWML2}4:1:P16;, MCHP_MASTERLINK=SAME70_AFEC_dvpt_R2010a/Microchip Master, invert_PWMH0=off, invert_PWML0=off, invert_PWMH1=off, invert_PWML1=off, invert_PWMH2=off, invert_PWML2=off, invert_PWMH3=off, invert_PWML3=off, InitPeriod_s=1e-3, InitDutyCycle_s=0.5e-3, InitDeadTimeH_s=0e-6, InitDeadTimeL_s=0e-6, InitEventLine0_ComparatorValue_s=1e-3, InitEventLine1_ComparatorValue_s=[], BlockInput_VectorScalar=Vectors (grouped by function), BlockInput_Period=a Floating Point input within range [0 1], BlockInput_DutyCycle=a Floating Point input within range [0 1], BlockInput_DeadTime=Not a block input, BlockInput_OutputOverride=Not a block input, Fault_FPV0=Not forced, Fault_FPV1=Not forced, Fault_FPV2=Not forced, Fault_FPV3=Not forced, Fault_Input0=does nothing, Fault_Input0_FFIL=off, Fault_Input1=does nothing, Fault_Input1_FFIL=off, Fault_Input2=does nothing, Fault_Input2_FFIL=on, Fault_Input3=does nothing, Fault_Input3_FFIL=off, Fault_Input4=does nothing, Fault_Input4_FFIL=on, Fault_Input5=does nothing, Fault_Input5_FFIL=on, Fault_Input6=does nothing, Fault_Input6_FFIL=on, Fault_Input7=does nothing, Fault_Input7_FFIL=on}
      mask prompts: PWMx "Select Pulse Width Modulation (PWM) Controller :"; MaxPeriod_s "Max period (s)  PWM{1 2 3}max0 = 2^15.19 (37500) for 0.001s"; PWM0_pinH0 "PWMH0"; PWM0_pinL0 "PWML0"; PWM0_pinH1 "PWMH1"; PWM0_pinL1 "PWML1"; PWM0_pinH2 "PWMH2"; PWM0_pinL2 "PWML2"; PWM0_pinH3 "PWMH3"; PWM0_pinL3 "PWML3"; PWM1_pinH0 "PWMH0"; PWM1_pinL0 "PWML0"; PWM1_pinH1 "PWMH1"; PWM1_pinL1 "PWML1"; PWM1_pinH2 "PWMH2"; PWM1_pinL2 "PWML2"; PWM1_pinH3 "PWMH3"; PWM1_pinL3 "PWML3"; PWM_Centered "Center aligned (left aligned otherwise)"; PWM_SyncWithPWM0 "Synchronized (with PWM0)"; PushPull_Mode "Push-Pull Mode"; SampleTime "Block output sample time"; invert_PWMH0 "Invert PWMH0"; invert_PWML0 "Invert PWML0"; invert_PWMH1 "Invert PWMH1"; invert_PWML1 "Invert PWML1"; invert_PWMH2 "Invert PWMH2"; invert_PWML2 "Invert PWML2"; invert_PWMH3 "Invert PWMH3"; invert_PWML3 "Invert PWML3"; InitPeriod_s "Initial Period (in s)"; InitDutyCycle_s "Initial Duty Cycle (in s)"; InitDeadTimeH_s "Initial Dead-time for PWMHx (in s)"; InitDeadTimeL_s "Initial Dead-time for PWMLx (in s)"; InitEventLine0_ComparatorValue_s "Event Line 0 Trigger(s). Up to 8 comparator values (in s)"; InitEventLine1_ComparatorValue_s "Event Line 1 Trigger(s). Up to 8 comparator values (in s)"; BlockInput_VectorScalar "Block input format"; BlockInput_Period "Period"; BlockInput_DutyCycle "Duty Cycle"; BlockInput_DeadTime "Dead Time"; BlockInput_OutputOverride "Output Override"; Fault_FPV0 "PWM0 force on fault:"; Fault_FPV1 "PWM1 force on fault:"; Fault_FPV2 "PWM2 force on fault:"; Fault_FPV3 "PWM3 force on fault:"; Fault_Input0 "PWMFI0 input pin"; Fault_Input0_FFIL "PWMFI0 is filtered for glitches"; Fault_Input1 "PWMFI1 input pin"; Fault_Input1_FFIL "PWMFI1 is filtered for glitches"; Fault_Input2 "PWMFI2 input pin"; Fault_Input2_FFIL "PWMFI2 is filtered for glitches"; Fault_Input3 "Oscillator fault"; Fault_Input3_FFIL "Oscillator fault is filtered for glitches"; Fault_Input4 "Analog to Digital Converter (AFEC0)"; Fault_Input4_FFIL "Analog to Digital Converter(AFEC0) is filtered for glitches"; Fault_Input5 "Analog to Digital Converter (AFEC1)"; Fault_Input5_FFIL "Analog to Digital Converter (AFEC1) s filtered for glitches"; Fault_Input6 "Analog Comparator (ACC)"; Fault_Input6_FFIL "Analog Comparator is filtered for glitches"; Fault_Input7 "Timer 0"; Fault_Input7_FFIL "Timer 0 is filtered for glitches"
      mask help:
      | Set-up Pulse Width Modulation (PWM) peripheral.
      | A PWM Channel is configured when one output pin is set (High and/or Low side).
      |
      | The main tab parameters are applied to all channel declared by this block instance.
      | Multiple instance of the PWM block is possible allowing to configure others PWM channels with different settings.
      |
      | Impossible set-up are detected and reported at compilation time. For example PWM0 from controller 0 set-up in two blocks with different setting for the initial period.
      mask init:
      | MCHP_PWM_SAM7x_Callback(gcbh,'INITIALISATION');
      settings: CopyFcn=MCHP_PWM_SAM7x_Callback(gcbh,'CopyFcn');  PreSaveFcn=MCHP_Fun.PreSaveFcn_DynamicOptions(gcbh);  OpenFcn=MCHP_PWM_SAM7x_Callback(gcbh,'OPEN');
      mask TypeOptions PWMx: PWM Controller 0 | PWM Controller 1
      mask Callback PWMx: MCHP_PWM_SAM7x_Callback(gcbh,'UpdateGUI');
      mask TypeOptions PWM0_pinH0: Dynamic Options
      mask Callback PWM0_pinH0: MCHP_PWM_SAM7x_Callback(gcbh,'UpdateGUI');
      mask TypeOptions PWM0_pinL0: Dynamic Options
      mask Callback PWM0_pinL0: MCHP_PWM_SAM7x_Callback(gcbh,'UpdateGUI');
      mask TypeOptions PWM0_pinH1: Dynamic Options
      mask Callback PWM0_pinH1: MCHP_PWM_SAM7x_Callback(gcbh,'UpdateGUI');
      mask TypeOptions PWM0_pinL1: Dynamic Options
      mask Callback PWM0_pinL1: MCHP_PWM_SAM7x_Callback(gcbh,'UpdateGUI');
      mask TypeOptions PWM0_pinH2: Dynamic Options
      mask Callback PWM0_pinH2: MCHP_PWM_SAM7x_Callback(gcbh,'UpdateGUI');
      mask TypeOptions PWM0_pinL2: Dynamic Options
      mask Callback PWM0_pinL2: MCHP_PWM_SAM7x_Callback(gcbh,'UpdateGUI');
      mask TypeOptions PWM0_pinH3: Dynamic Options
      mask Callback PWM0_pinH3: MCHP_PWM_SAM7x_Callback(gcbh,'UpdateGUI');
      mask TypeOptions PWM0_pinL3: Dynamic Options
      mask Callback PWM0_pinL3: MCHP_PWM_SAM7x_Callback(gcbh,'UpdateGUI');
      mask TypeOptions PWM1_pinH0: Dynamic Options
      mask Callback PWM1_pinH0: MCHP_PWM_SAM7x_Callback(gcbh,'UpdateGUI');
      mask TypeOptions PWM1_pinL0: Dynamic Options
      mask Callback PWM1_pinL0: MCHP_PWM_SAM7x_Callback(gcbh,'UpdateGUI');
      mask TypeOptions PWM1_pinH1: Dynamic Options
      mask Callback PWM1_pinH1: MCHP_PWM_SAM7x_Callback(gcbh,'UpdateGUI');
      mask TypeOptions PWM1_pinL1: Dynamic Options
      mask Callback PWM1_pinL1: MCHP_PWM_SAM7x_Callback(gcbh,'UpdateGUI');
      mask TypeOptions PWM1_pinH2: Dynamic Options
      mask Callback PWM1_pinH2: MCHP_PWM_SAM7x_Callback(gcbh,'UpdateGUI');
      mask TypeOptions PWM1_pinL2: Dynamic Options
      mask Callback PWM1_pinL2: MCHP_PWM_SAM7x_Callback(gcbh,'UpdateGUI');
      mask TypeOptions PWM1_pinH3: Dynamic Options
      mask Callback PWM1_pinH3: MCHP_PWM_SAM7x_Callback(gcbh,'UpdateGUI');
      mask TypeOptions PWM1_pinL3: Dynamic Options
      mask Callback PWM1_pinL3: MCHP_PWM_SAM7x_Callback(gcbh,'UpdateGUI');
      mask TypeOptions BlockInput_VectorScalar: Independent Scalar | Vectors (grouped by function)
      mask TypeOptions BlockInput_Period: Not a block input | a Uint raw input (PWMxmax variable represent max period) | a Floating Point input within range [0 1] | a Floating Point input within range [-1 1] | a Floating Point input with physical scaling in (s)
      mask TypeOptions BlockInput_DutyCycle: Not a block input | a Uint raw input (PWMxmax variable represent max period) | a Floating Point input within range [0 1] | a Floating Point input within range [-1 1] | a Floating Point input with physical scaling in (s)
      mask TypeOptions BlockInput_DeadTime: Not a block input | a Uint raw input (PWMxmax variable represent max period) | a Floating Point input within range [0 1] | a Floating Point input within range [-1 1] | a Floating Point input with physical scaling in (s)
      mask Callback BlockInput_DeadTime: MCHP_PWM_SAM7x_Callback(gcbh,'UpdateGUI');
      mask TypeOptions BlockInput_OutputOverride: Not a block input | Boolean Input
      mask TypeOptions Fault_FPV0: Not forced | --- Z if High Impedance --- | PWM H/L -> 00 | PWM H/L -> ZZ | PWM H/L -> 11 | PWM H/L -> 01 | PWM H/L -> 10 | PWM H/L -> 1Z | PWM H/L -> 0Z | PWM H/L -> Z1 | PWM H/L -> Z0 | --- one side only --- | PWM H -> 0- | PWM H -> 1- | PWM H -> Z- | PWM L -> -0 | PWM L -> -1 | PWM L -> -Z
      mask Callback Fault_FPV0: MCHP_PWM_SAM7x_Callback(gcbh,'UpdateGUI');
      mask TypeOptions Fault_FPV1: Not forced | --- Z if High Impedance --- | PWM H/L -> 00 | PWM H/L -> ZZ | PWM H/L -> 11 | PWM H/L -> 01 | PWM H/L -> 10 | PWM H/L -> 1Z | PWM H/L -> 0Z | PWM H/L -> Z1 | PWM H/L -> Z0 | --- one side only --- | PWM H -> 0- | PWM H -> 1- | PWM H -> Z- | PWM L -> -0 | PWM L -> -1 | PWM L -> -Z
      mask Callback Fault_FPV1: MCHP_PWM_SAM7x_Callback(gcbh,'UpdateGUI');
      mask TypeOptions Fault_FPV2: Not forced | --- Z if High Impedance --- | PWM H/L -> 00 | PWM H/L -> ZZ | PWM H/L -> 11 | PWM H/L -> 01 | PWM H/L -> 10 | PWM H/L -> 1Z | PWM H/L -> 0Z | PWM H/L -> Z1 | PWM H/L -> Z0 | --- one side only --- | PWM H -> 0- | PWM H -> 1- | PWM H -> Z- | PWM L -> -0 | PWM L -> -1 | PWM L -> -Z
      mask Callback Fault_FPV2: MCHP_PWM_SAM7x_Callback(gcbh,'UpdateGUI');
      mask TypeOptions Fault_FPV3: Not forced | --- Z if High Impedance --- | PWM H/L -> 00 | PWM H/L -> ZZ | PWM H/L -> 11 | PWM H/L -> 01 | PWM H/L -> 10 | PWM H/L -> 1Z | PWM H/L -> 0Z | PWM H/L -> Z1 | PWM H/L -> Z0 | --- one side only --- | PWM H -> 0- | PWM H -> 1- | PWM H -> Z- | PWM L -> -0 | PWM L -> -1 | PWM L -> -Z
      mask Callback Fault_FPV3: MCHP_PWM_SAM7x_Callback(gcbh,'UpdateGUI');
      mask TypeOptions Fault_Input0: does nothing | trig a fault on level high | trig a fault on level low
      mask TypeOptions Fault_Input1: does nothing | trig a fault on level high | trig a fault on level low
      mask Callback Fault_Input1: MCHP_PWM_SAM7x_Callback(gcbh,'UpdateGUI');
      mask TypeOptions Fault_Input2: does nothing | trig a fault on level high | trig a fault on level low
      mask Callback Fault_Input2: MCHP_PWM_SAM7x_Callback(gcbh,'UpdateGUI');
      mask TypeOptions Fault_Input3: does nothing | trig a fault
      mask Callback Fault_Input3: MCHP_PWM_SAM7x_Callback(gcbh,'UpdateGUI');
      mask TypeOptions Fault_Input4: does nothing | trig a fault
      mask Callback Fault_Input4: MCHP_PWM_SAM7x_Callback(gcbh,'UpdateGUI');
      mask TypeOptions Fault_Input5: does nothing | trig a fault
      mask TypeOptions Fault_Input6: does nothing | trig a fault
      mask Callback Fault_Input6: MCHP_PWM_SAM7x_Callback(gcbh,'UpdateGUI');
      mask TypeOptions Fault_Input7: does nothing | trig a fault
      mask Callback Fault_Input7: MCHP_PWM_SAM7x_Callback(gcbh,'UpdateGUI');
      mask Display:
      | fprintf(['PWM SAMx7\n' PWMx(4:end)]);
      | port_label('input',1,'Period');
      | port_label('input',2,'DutyCycle[0 1 2]');
  PWM SAM7x Output Override : S-Function  Priority=-2000  InitFcn=MCHP_PWM_SAM7x_Override_Callback(gcbh,'InitFcn');  FunctionName=MCHP_PWM_SAM7x_Override  Parameters=MCHP_PWM_SAM7x_Override_Callback(gcbh,'S_INPUT'),MCHP_PWM_SAM7x_Override_Callback(gcbh,'S_OUTPUT'),MCHP_PWM_SAM7x_Override_Callback(gcbh,'S_INPUT_Size'),MCHP_PWM_SAM7x_Override_Callback(gcbh,'S_OUTPUT_Size'),MCHP_PWM_SAM7x_Override_Callback(gcbh,'S_ListCustomDatatype'),SampleTime,0  EnableBusSupport=off  mask(PWM Override for SAMx7){PWMx=PWM Controller 0, SampleTime=-1, S_INPUT=[-1], S_INPUT_Size=[3], S_OUTPUT=[], S_OUTPUT_Size=[], S_ListCustomDatatype=S.S_ListCustomDatatype={};, MCHP_MASTERLINK=SAMx7_PWM_Override_R2014b/Microchip Master, Init_PWM_OS=0x0000, Init_PWM_OOV=0x0000, Input_PWM_OS=on, Input_PWM_OS_off=off, Input_PWM_OSS=off, Input_PWM_OSS_off=off, Input_PWM_OSSUPD=off, Input_PWM_OSSUPD_off=off, Input_PWM_OSC=off, Input_PWM_OSC_off=off, Input_PWM_OSCUPD=off, Input_PWM_OSCUPD_off=off, Input_PWM_OOV=on}
      mask prompts: PWMx "Select Pulse Width Modulation (PWM) Controller :"; SampleTime "Block sample time"; Init_PWM_OS "Initial PWM output selection (bitewise 1 override; 0 PWM)"; Init_PWM_OOV "Initial PWM override output value (bitewise)"; Input_PWM_OS "PWM output selection is a block input (bitewise 1 override; 0 PWM)"; Input_PWM_OS_off "PWM output selection is a block input (bitewise 1 override; 0 PWM)"; Input_PWM_OSS "PWM output selection set to override value (bitewise 1 set override; 0 no action)"; Input_PWM_OSS_off "PWM output selection set to override value (bitewise 1 set override; 0 no action)"; Input_PWM_OSSUPD "Synchronize set to override with PWM period"; Input_PWM_OSSUPD_off "Synchronize set to override with PWM period"; Input_PWM_OSC "PWM output selection set to PWM (bitewise 1 set PWM; 0 no action)"; Input_PWM_OSC_off "PWM output selection set to PWM (bitewise 1 set PWM; 0 no action)"; Input_PWM_OSCUPD "Synchronize set to PWM with PWM period"; Input_PWM_OSCUPD_off "Synchronize set to PWM with PWM period"; Input_PWM_OOV "PWM override output value is a block input (bitewise)"
      mask help:
      | Initial value and block input map to peripehral override register.
      | bits [0:3] map to PWM High side output ; bits [16:19] map to PWM Low side output:
      |
      | H0 is at position 0 (LSB)
      | L0 is at position 16.
      | [x x x x x x x x x x x x L3 L2 L1 L0 x x x x x x x x x x x x H3 H2 H1 H0]
      |
      | Override can be synchronized with to the next PWM period.
      mask init:
      | MCHP_PWM_SAM7x_Override_Callback(gcbh,'INITIALISATION');
      settings: CopyFcn=MCHP_PWM_SAM7x_Override_Callback(gcbh,'CopyFcn');  PreSaveFcn=MCHP_Fun.PreSaveFcn_DynamicOptions(gcbh);  OpenFcn=MCHP_PWM_SAM7x_Override_Callback(gcbh,'OPEN');
      mask TypeOptions PWMx: PWM Controller 0 | PWM Controller 1
      mask Callback Input_PWM_OS: MCHP_PWM_SAM7x_Override_Callback(gcbh,'UpdateGUI');
      mask Callback Input_PWM_OSS: MCHP_PWM_SAM7x_Override_Callback(gcbh,'UpdateGUI');
      mask Callback Input_PWM_OSSUPD: MCHP_PWM_SAM7x_Override_Callback(gcbh,'UpdateGUI');
      mask Callback Input_PWM_OSC: MCHP_PWM_SAM7x_Override_Callback(gcbh,'UpdateGUI');
      mask Callback Input_PWM_OSCUPD: MCHP_PWM_SAM7x_Override_Callback(gcbh,'UpdateGUI');
      mask Callback Input_PWM_OOV: MCHP_PWM_SAM7x_Override_Callback(gcbh,'UpdateGUI');
      mask Display:
      | fprintf(['PWM Override SAMx7\n' PWMx(4:end)]);
      | port_label('input',1,'Override set/clr');
      | port_label('input',2,'output values');
  PWM TCC : S-Function  LoadFcn=MCHP_Fun.Load_EvalIn_ws(gcbh);  InitFcn=MCHP_TCC_PWM_Callback(gcb,'InitFcn');  FunctionName=MCHP_TCC_PWM  Parameters=MCHP_TCC_PWM_Callback(gcbh,'S_INPUT'),MCHP_TCC_PWM_Callback(gcbh,'S_OUTPUT'),MCHP_TCC_PWM_Callback(gcbh,'S_INPUT_Size'),MCHP_TCC_PWM_Callback(gcbh,'S_OUTPUT_Size'),MCHP_TCC_PWM_Callback(gcbh,'S_ListCustomDatatype'),SampleTime,0  EnableBusSupport=off  mask(PWM - TCC){TCCREF=TCC 0, WAVE_choice=Left aligned PWM, MaxPeriod_s=1e-3, OTMX=Default, WO0=Dynamic Options, WO0_TXT=PA08 / Pin[33], WO1=Dynamic Options, WO1_TXT=PA09 / Pin[34], WO2=Dynamic Options, WO2_TXT=PA10 / Pin[35], WO3=Dynamic Options, WO3_TXT=Not Used, WO4=Dynamic Options, WO4_TXT=PA16 / Pin[66], WO5=Dynamic Options, WO5_TXT=PA17 / Pin[67], WO6=Dynamic Options, WO6_TXT=PA18 / Pin[68], WO7=Dynamic Options, WO7_TXT=Not Used, info=0, evalin_ws=PWM0max=MCHP_Fun.Hex2num('40F869F000000000');PWM0max=MCHP_Fun.Hex2num('40F869F000000000');PWM0max=MCHP_Fun.Hex2num('40F869F000000000');, SampleTime=.001, MCHP_PORT={PWM0_H0}{TCC0_WO0}5:1:P8;{PWM0_H1}{TCC0_WO1}5:1:P9;{PWM0_H2}{TCC0_WO2}5:1:P10;{PWM0_L0}{TCC0_WO4}5:1:P16;{PWM0_L1}{TCC0_WO5}5:1:P17;{PWM0_L2}{TCC0_WO6}5:1:P18;, MCHP_MASTERLINK=SAME5x_PIM_MCLV2_ADC_R2014b/Microchip Master, INVEN_WO0=off, INVEN_WO1=off, INVEN_WO2=off, INVEN_WO3=off, INVEN_WO4=off, INVEN_WO5=off, INVEN_WO6=off, INVEN_WO7=off, SWAP_PWM0=off, SWAP_PWM1=off, SWAP_PWM2=off, SWAP_PWM3=off, POL_PWM0=off, POL_PWM1=off, POL_PWM2=off, POL_PWM3=off, POL_PWM4=off, POL_PWM5=off, InitPeriod_s=1e-3, InitDutyCycle_s=0.5e-3, InitDeadTimeH_s=1e-6, InitDeadTimeL_s=1e-6, InitOutputOverride=0, InitOutputOverride_val=0, BlockInput_VectorScalar=Vectors (grouped by function), BlockInput_Period=Not a block input, BlockInput_DutyCycle=a Floating Point input within range [-1 1], BlockInput_DeadTime=Not a block input, BlockInput_OutputOverride=Not a block input}
      mask prompts: TCCREF "Select Pulse Width Modulation (PWM) Controller"; WAVE_choice "Generate signal"; MaxPeriod_s "Max period (s)  PWM0max = 2^16.61 (99999) for 0.001s"; OTMX "Output Mapping matrix"; WO0 "Pin WO0 - PWM0_H0"; WO0_TXT "output pin WO0"; WO1 "Pin WO1 - PWM0_H1"; WO1_TXT "output pin WO1"; WO2 "Pin WO2 - PWM0_H2"; WO2_TXT "output pin WO2"; WO3 "Pin WO3 - PWM0_H3"; WO3_TXT "output pin WO3"; WO4 "Pin WO4 - PWM0_L0"; WO4_TXT "output pin WO4"; WO5 "Pin WO5 - PWM0_L1"; WO5_TXT "output pin WO5"; WO6 "Pin WO6 - PWM0_L2"; WO6_TXT "output pin WO6"; WO7 "Pin WO7 - PWM0_L3"; WO7_TXT "output pin WO7"; SampleTime "Sample Time"; INVEN_WO0 "Invert WO0 - PWM0_H0 output"; INVEN_WO1 "Invert WO1 - PWM0_H1 output"; INVEN_WO2 "Invert WO2 - PWM0_H2 output"; INVEN_WO3 "Invert WO3 output"; INVEN_WO4 "Invert WO4 - PWM0_L0 output"; INVEN_WO5 "Invert WO5 - PWM0_L1 output"; INVEN_WO6 "Invert WO6 - PWM0_L2 output"; INVEN_WO7 "Invert WO7 output"; SWAP_PWM0 "SWAP PWM0 High-Low side"; SWAP_PWM1 "SWAP PWM1 High-Low side"; SWAP_PWM2 "SWAP PWM2 High-Low side"; SWAP_PWM3 "SWAP PWM3 High-Low side"; POL_PWM0 "Reverse PWM0 polarity"; POL_PWM1 "Reverse PWM1 polarity"; POL_PWM2 "Reverse PWM2 polarity"; POL_PWM3 "Reverse PWM3 polarity"; POL_PWM4 "Reverse PWM4 polarity"; POL_PWM5 "Reverse PWM5 polarity"; InitPeriod_s "Initial Period (in s)"; InitDutyCycle_s "Initial Duty Cycle (in s)"; InitDeadTimeH_s "Initial Dead-time for PWMHx (in s)"; InitDeadTimeL_s "Initial Dead-time for PWMLx (in s)"; InitOutputOverride "Initial PIN WOx Output Override ; bitewise (PATT LSB: 0 : 1 is activated)"; InitOutputOverride_val "Initial PIN WOx Output Override value ; bitewise (PATT MSB)"; BlockInput_VectorScalar "Block input format"; BlockInput_Period "Period"; BlockInput_DutyCycle "Duty Cycle"; BlockInput_DeadTime "Dead Time"; BlockInput_OutputOverride "Override Output"
      mask help: PWM peripheral for SAMD/E5x and SAMx2 based on TCC.
      mask init:
      | MCHP_TCC_PWM_Callback(gcbh,'INITIALISATION');
      settings: CopyFcn=MCHP_Fun.BlockUpdate(gcbh);  DeleteFcn=MCHP_TCC_PWM_Callback(gcbh,'DeleteFcn');  PreSaveFcn=MCHP_Fun.PreSaveFcn_DynamicOptions(gcbh);  OpenFcn=MCHP_TCC_PWM_Callback(gcb,'OPEN');
      mask TypeOptions TCCREF: TCC 0 | TCC 1 | TCC 2 | TCC 3 | TCC 4
      mask Callback TCCREF: MCHP_TCC_PWM_Callback(gcbh,'UpdateGUI');
      mask TypeOptions WAVE_choice: Left aligned PWM | Center aligned PWM
      mask TypeOptions OTMX: Default | Variant 1 | Variant 2 | Variant 3
      mask Callback OTMX: MCHP_TCC_PWM_Callback(gcbh,'UpdateGUI');
      mask TypeOptions WO0: Dynamic Options
      mask TypeOptions WO1: Dynamic Options
      mask TypeOptions WO2: Dynamic Options
      mask TypeOptions WO3: Dynamic Options
      mask TypeOptions WO4: Dynamic Options
      mask TypeOptions WO5: Dynamic Options
      mask TypeOptions WO6: Dynamic Options
      mask TypeOptions WO7: Dynamic Options
      mask TypeOptions BlockInput_VectorScalar: Independent Scalar | Vectors (grouped by function)
      mask TypeOptions BlockInput_Period: Not a block input | a Uint raw input (PWMxmax variable represent max period) | a Floating Point input within range [0 1] | a Floating Point input within range [-1 1] | a Floating Point input with physical scaling in (s)
      mask TypeOptions BlockInput_DutyCycle: Not a block input | a Uint raw input (PWMxmax variable represent max period) | a Floating Point input within range [0 1] | a Floating Point input within range [-1 1] | a Floating Point input with physical scaling in (s)
      mask TypeOptions BlockInput_DeadTime: Not a block input | a Uint raw input (PWMxmax variable represent max period) | a Floating Point input within range [0 1] | a Floating Point input within range [-1 1] | a Floating Point input with physical scaling in (s)
      mask TypeOptions BlockInput_OutputOverride: Not a block input | --- IMMEDIATE --- |  RAW PATT register ; 8 LSB is override active ; 8MSB is out val (Imm) |  Override Activation & pin ouptut value block inputs (Imm) |  Override Activation only (default output val) (Imm) | ---SYNC with PWM period --- |  RAW PATT register ; 8 LSB is override active ; 8MSB is out val |  Override Activation & pin ouptut value block inputs |  Override Activation only (default output val)
      mask Display:
      | fprintf(['PWM\nTCC' TCCREF(4:end)]);
      | port_label('input',1,'DutyCycle[0 1 2]');
  PWM_HS_FEP : S-Function  Priority=-2000  LoadFcn=MCHP_Fun.Load_EvalIn_ws(gcbh);  InitFcn=MCHP_PWM_HS_FEP_Callback(gcbh,'InitFcn');  FunctionName=MCHP_PWM_HS_FEP  Parameters=MCHP_PWM_HS_FEP_Callback(gcbh,'S_INPUT'),MCHP_PWM_HS_FEP_Callback(gcbh,'S_OUTPUT'),MCHP_PWM_HS_FEP_Callback(gcbh,'S_INPUT_Size'),MCHP_PWM_HS_FEP_Callback(gcbh,'S_OUTPUT_Size'),MCHP_PWM_HS_FEP_Callback(gcbh,'S_ListCustomDatatype'),SampleTime,0  EnableBusSupport=off  mask(PWM High-Speed Fine-Edge-Placement){PWMx_MODSEL=Edge Aligned - Duty Cycle and Phase Shift, PWMx_CLKSEL=Use divider circuit, PWM_ClockResolution_DIVSEL=Dynamic Options, PWM_ClockResolution_DIVSEL_TXT=auto, PWM_ClockResolution_FSCL=Dynamic Options, PWM_ClockResolution_FSCL_TXT=Resol: 0.04878(us)  -  MaxPer: 0.0032(s), PWM_ClockResolution_NoScaling=Dynamic Options, PWM_ClockResolution_NoScaling_TXT=Resol: 0.006098(us)  -  MaxPer: 0.0004(s), MaxPeriod_s=50e-6, InitPeriode_s=50e-6, InitDutyCycleP_s=0, InitDutyCycleS_s=10e-6, InitPhase_s=-1, evalin_ws='', SampleTime=-1, S_INPUT=[-1], S_INPUT_Size=[3], S_OUTPUT=[], S_OUTPUT_Size=[], S_ListCustomDatatype=S.S_ListCustomDatatype={};, MCHP_USER_INTERRUPTS=0, MCHP_PORT={PWMH1 }{PWMH1}32:4:B14;{PWMH2 }{PWMH2}32:4:B12;{PWMH3 }{PWMH3}32:4:B10;{PWML1}{PWML1}32:4:B15;{PWML2}{PWML2}32:4:B13;{PWML3}{PWML3}32:4:B11;, MCHP_MASTERLINK=dsPIC33CK_PWM_R2014b/Microchip Master, MCHP_CRC=4691235, INFO=, PWMx_PMOD=Complementary, PWM1_HL=PWMxH & PWMxL output enabled, PWM1_swap=off, PWM1H_pol=off, PWM1L_pol=off, PWM2_HL=PWMxH & PWMxL output enabled, PWM2_swap=off, PWM2H_pol=off, PWM2L_pol=off, PWM3_HL=PWMxH & PWMxL output enabled, PWM3_swap=off, PWM3H_pol=off, PWM3L_pol=off, PWM4_HL=not used, PWM4_swap=off, PWM4H_pol=off, PWM4L_pol=off, PWM5_HL=not used, PWM5_swap=off, PWM5H_pol=off, PWM5L_pol=off, PWM6_HL=not used, PWM6_swap=off, PWM6H_pol=off, PWM6L_pol=off, PWM7_HL=not used, PWM7_swap=off, PWM7H_pol=off, PWM7L_pol=off, PWM8_HL=not used, PWM8_swap=off, PWM8H_pol=off, PWM8L_pol=off, PWM9_HL=not used, PWM9_swap=off, PWM9H_pol=off, PWM9L_pol=off, PWM10_HL=not used, PWM10_swap=off, PWM10H_pol=off, PWM10L_pol=off, PWM11_HL=not used, PWM11_swap=off, PWM11H_pol=off, PWM11L_pol=off, PWM12_HL=not used, PWM12_swap=off, PWM12H_pol=off, PWM12L_pol=off, PWM1_ShowTrig=off, PWM1_Init_PGxTRIGABC_s=[0 -1 -1 ], PWM1_ADTRxEN1=ADC Trigger 1, PWM1_ADTRxEN2=none, PWM1_ADTRxEN3=none, PWM2_ShowTrig=off, PWM2_Init_PGxTRIGABC_s=[-1 -1 -1], PWM2_ADTRxEN1=none, PWM2_ADTRxEN2=none, PWM2_ADTRxEN3=none, PWM3_ShowTrig=off, PWM3_Init_PGxTRIGABC_s=[-1 -1 -1], PWM3_ADTRxEN1=none, PWM3_ADTRxEN2=none, PWM3_ADTRxEN3=none, PWM4_ShowTrig=off, PWM4_Init_PGxTRIGABC_s=[-1 -1 -1], PWM4_ADTRxEN1=none, PWM4_ADTRxEN2=none, PWM4_ADTRxEN3=none, PWM5_ShowTrig=off, PWM5_Init_PGxTRIGABC_s=[-1 -1 -1], PWM5_ADTRxEN1=none, PWM5_ADTRxEN2=none, PWM5_ADTRxEN3=none, PWM6_ShowTrig=off, PWM6_Init_PGxTRIGABC_s=[-1 -1 -1], PWM6_ADTRxEN1=none, PWM6_ADTRxEN2=none, PWM6_ADTRxEN3=none, PWM7_ShowTrig=off, PWM7_Init_PGxTRIGABC_s=[-1 -1 -1], PWM7_ADTRxEN1=none, PWM7_ADTRxEN2=none, PWM7_ADTRxEN3=none, PWM8_ShowTrig=off, PWM8_Init_PGxTRIGABC_s=[-1 -1 -1], PWM8_ADTRxEN1=none, PWM8_ADTRxEN2=none, PWM8_ADTRxEN3=none, BlockInput_VectorScalar=Independant Scalar, BlockInput_Period=Not a block input, BlockInput_DutyCycle=a Uint raw input (PWMxmax variable represent max period), BlockInput_PhaseShift=Not a block input, BlockInput_SEVTCMP=Not a block input, BlockInput_TRIGx=Not a block input, BlockInput_DeadTime=Not a block input, BlockOutput_FaultDisabled=off, BlockOutput_Fault=on, DTC=Positive dead time (ensure period of time with PWM_H and PWM_L disasserted), FLTSRC1_DTCMP=Dynamic Options, FLTSRC1_DTCMP_TXT=<empty>, FLTSRC2_DTCMP=Dynamic Options, FLTSRC2_DTCMP_TXT=<empty>, FLTSRC3_DTCMP=Dynamic Options, FLTSRC3_DTCMP_TXT=<empty>, FLTSRC4_DTCMP=Dynamic Options, FLTSRC4_DTCMP_TXT=<empty>, FLTSRC5_DTCMP=Dynamic Options, FLTSRC5_DTCMP_TXT=<empty>, FLTSRC6_DTCMP=Dynamic Options, FLTSRC6_DTCMP_TXT=<empty>, FLTSRC7_DTCMP=Dynamic Options, FLTSRC7_DTCMP_TXT=<empty>, FLTSRC8_DTCMP=Dynamic Options, FLTSRC8_DTCMP_TXT=<empty>, FLTSRC9_DTCMP=Dynamic Options, FLTSRC9_DTCMP_TXT=<empty>, FLTSRC10_DTCMP=Dynamic Options, FLTSRC10_DTCMP_TXT=<empty>, FLTSRC11_DTCMP=Dynamic Options, FLTSRC11_DTCMP_TXT=<empty>, FLTSRC12_DTCMP=Dynamic Options, FLTSRC12_DTCMP_TXT=<empty>, DeadTime_s=2e-6, DeadTimeAlt_s=2e-6, DeadTimeComp_s=0, FLTMODx=Disabled, FLTSRCx=Dynamic Options, FLTSRCx_TXT=<empty>, FLTDATx=PWM H/L -> 11, CLMODx=Disabled, CLSRCx=Dynamic Options, CLSRCx_TXT=<empty>, CLDATx=PWM H/L -> 00, FLTLEBENx=off, CLLEBENx=off, LeadEdgeBlkPer_s=5e-7, PHRx=off, PHFx=off, PLRx=off, PLFx=off}
      mask prompts: PWMx_MODSEL "PWM set with Period and"; PWMx_CLKSEL "Clock source :"; PWM_ClockResolution_DIVSEL "Clock source resolution : [PWM res 6.098(ns) => periode up to 400(us) ]"; PWM_ClockResolution_DIVSEL_TXT "<empty>"; PWM_ClockResolution_FSCL "PWM clock Resolution :"; PWM_ClockResolution_FSCL_TXT "<empty>"; PWM_ClockResolution_NoScaling "PWM clock Resolution :"; PWM_ClockResolution_NoScaling_TXT "unused"; MaxPeriod_s "Max Period (s) : PWM1max=PWM2max=PWM3max=8199 (13bits)  represent 50(us)"; InitPeriode_s "Initial Period (s) :"; InitDutyCycleP_s "Initial Duty-Cycle (s) :"; InitDutyCycleS_s "Initial second half Duty Cycle (s)"; InitPhase_s "Initial Phase-Shift (s) :"; SampleTime "Block output sample time"; INFO "Infos"; PWMx_PMOD "High/Low side Mode :"; PWM1_HL "PWM 1 Channel"; PWM1_swap "Swap PWM1_H and PWM1_L"; PWM1H_pol "invert PWM1_H output polarity ( B14 [1] active low )"; PWM1L_pol "invert PWM1_L output polarity ( B15 [3] active low )"; PWM2_HL "PWM 2 Channel"; PWM2_swap "Swap PWM2_H and PWM2_L"; PWM2H_pol "invert PWM2_H output polarity ( B12 [78] active low )"; PWM2L_pol "invert PWM2_L output polarity ( B13 [80] active low )"; PWM3_HL "PWM 3 Channel"; PWM3_swap "Swap PWM3_H and PWM3_L"; PWM3H_pol "invert PWM3_H output polarity ( B10 [75] active low )"; PWM3L_pol "invert PWM3_L output polarity ( B11 [76] active low )"; PWM4_HL "PWM 4 Channel"; PWM4_swap "Swap PWM4_H and PWM4_L"; PWM4H_pol "invert PWM4_H output polarity ( D1 [73] active low )"; PWM4L_pol "invert PWM4_L output polarity ( D0 [74] active low )"; PWM5_HL "PWM 5 Channel"; PWM5_swap "Swap PWM5_H and PWM5_L"; PWM5H_pol "invert PWM5_H output polarity ( C4 [63] active low )"; PWM5L_pol "invert PWM5_L output polarity ( C5 [65] active low )"; PWM6_HL "PWM 6 Channel"; PWM6_swap "Swap PWM6_H and PWM6_L"; PWM6H_pol "invert PWM6_H output polarity ( C14 [7] active low )"; PWM6L_pol "invert PWM6_L output polarity ( C15 [8] active low )"; PWM7_HL "PWM 7 Channel"; PWM7_swap "Swap PWM7_H and PWM7_L"; PWM7H_pol "invert PWM7_H output polarity ( C10 [66] active low )"; PWM7L_pol "invert PWM7_L output polarity ( C11 [67] active low )"; PWM8_HL "PWM 8 Channel"; PWM8_swap "Swap PWM8_H and PWM8_L"; PWM8H_pol "invert PWM8_H output polarity ( C12 [5] active low )"; PWM8L_pol "invert PWM8_L output polarity ( C13 [6] active low )"; PWM9_HL "<empty>"; PWM9_swap "<empty>"; PWM9H_pol "<empty>"; PWM9L_pol "<empty>"; PWM10_HL "<empty>"; PWM10_swap "<empty>"; PWM10H_pol "<empty>"; PWM10L_pol "<empty>"; PWM11_HL "<empty>"; PWM11_swap "<empty>"; PWM11H_pol "<empty>"; PWM11L_pol "<empty>"; PWM12_HL "<empty>"; PWM12_swap "<empty>"; PWM12H_pol "<empty>"; PWM12L_pol "<empty>"; PWM1_ShowTrig "Show Trigs for PWM 1"; PWM1_Init_PGxTRIGABC_s "PWM 1 TRIG A, B , C initial value (s) vector, -1 for not used"; PWM1_ADTRxEN1 "PWM 1 TRIG A is source for :"; PWM1_ADTRxEN2 "PWM 1 TRIG B is source for :"; PWM1_ADTRxEN3 "PWM 1 TRIG C is source for :"; PWM2_ShowTrig "Show Trigs for PWM 2"; PWM2_Init_PGxTRIGABC_s "PWM 2 TRIG A, B , C initial value (s) vector, -1 for not used"; PWM2_ADTRxEN1 "PWM 2 TRIG A is source for :"; PWM2_ADTRxEN2 "PWM 2 TRIG B is source for :"; PWM2_ADTRxEN3 "PWM 2 TRIG C is source for :"; PWM3_ShowTrig "Show Trigs for PWM 3"; PWM3_Init_PGxTRIGABC_s "PWM 3 TRIG A, B , C initial value (s) vector, -1 for not used"; PWM3_ADTRxEN1 "PWM 3 TRIG A is source for :"; PWM3_ADTRxEN2 "PWM 3 TRIG B is source for :"; PWM3_ADTRxEN3 "PWM 3 TRIG C is source for :"; PWM4_ShowTrig "Show Trigs for PWM 4"; PWM4_Init_PGxTRIGABC_s "PWM 4 TRIG A, B , C initial value (s) vector, -1 for not used"; PWM4_ADTRxEN1 "PWM 4 TRIG A is source for :"; PWM4_ADTRxEN2 "PWM 4 TRIG B is source for :"; PWM4_ADTRxEN3 "PWM 4 TRIG C is source for :"; PWM5_ShowTrig "Show Trigs for PWM 5"; PWM5_Init_PGxTRIGABC_s "PWM 5 TRIG A, B , C initial value (s) vector, -1 for not used"; PWM5_ADTRxEN1 "PWM 5 TRIG A is source for :"; PWM5_ADTRxEN2 "PWM 5 TRIG B is source for :"; PWM5_ADTRxEN3 "PWM 5 TRIG C is source for :"; PWM6_ShowTrig "Show Trigs for PWM 6"; PWM6_Init_PGxTRIGABC_s "PWM 6 TRIG A, B , C initial value (s) vector, -1 for not used"; PWM6_ADTRxEN1 "PWM 6 TRIG A is source for :"; PWM6_ADTRxEN2 "PWM 6 TRIG B is source for :"; PWM6_ADTRxEN3 "PWM 6 TRIG C is source for :"; PWM7_ShowTrig "Show Trigs for PWM 7"; PWM7_Init_PGxTRIGABC_s "PWM 7 TRIG A, B , C initial value (s) vector, -1 for not used"; PWM7_ADTRxEN1 "PWM 7 TRIG A is source for :"; PWM7_ADTRxEN2 "PWM 7 TRIG B is source for :"; PWM7_ADTRxEN3 "PWM 7 TRIG C is source for :"; PWM8_ShowTrig "Show Trigs for PWM 8"; PWM8_Init_PGxTRIGABC_s "PWM 8 TRIG A, B , C initial value (s) vector, -1 for not used"; PWM8_ADTRxEN1 "PWM 8 TRIG A is source for :"; PWM8_ADTRxEN2 "PWM 8 TRIG B is source for :"; PWM8_ADTRxEN3 "PWM 8 TRIG C is source for :"; BlockInput_VectorScalar "Block input format:"; BlockInput_Period "Period :"; BlockInput_DutyCycle "Duty-Cycle :"; BlockInput_PhaseShift "Phase-Shift :"; BlockInput_SEVTCMP "Master Time base event trigger :"; BlockInput_TRIGx "PWM Channel Primary/Secondary trigger :"; BlockInput_DeadTime "Dead Time :"; BlockOutput_FaultDisabled "PWM Fault State is a block Output"; BlockOutput_Fault "PWM Fault State is a block Output"; DTC "+++ Dead Time : +++"; FLTSRC1_DTCMP "Fault input pin for PWM 1"; FLTSRC1_DTCMP_TXT "<empty>"; FLTSRC2_DTCMP "Fault input pin for PWM 2"; FLTSRC2_DTCMP_TXT "<empty>"; FLTSRC3_DTCMP "Fault input pin for PWM 3"; FLTSRC3_DTCMP_TXT "<empty>"; FLTSRC4_DTCMP "Fault input pin for PWM 4"; FLTSRC4_DTCMP_TXT "<empty>"; FLTSRC5_DTCMP "Fault input pin for PWM 5"; FLTSRC5_DTCMP_TXT "<empty>"; FLTSRC6_DTCMP "Fault input pin for PWM 6"; FLTSRC6_DTCMP_TXT "<empty>"; FLTSRC7_DTCMP "Fault input pin for PWM 7"; FLTSRC7_DTCMP_TXT "<empty>"; FLTSRC8_DTCMP "Fault input pin for PWM 8"; FLTSRC8_DTCMP_TXT "<empty>"; FLTSRC9_DTCMP "<empty>"; FLTSRC9_DTCMP_TXT "<empty>"; FLTSRC10_DTCMP "<empty>"; FLTSRC10_DTCMP_TXT "<empty>"; FLTSRC11_DTCMP "<empty>"; FLTSRC11_DTCMP_TXT "<empty>"; FLTSRC12_DTCMP "<empty>"; FLTSRC12_DTCMP_TXT "<empty>"; DeadTime_s "Positive dead time on rising edge of PWM_H (s)"; DeadTimeAlt_s "Positive dead time on rising edge of PWM_L (s)"; DeadTimeComp_s "Dead Time Compensation value"; FLTMODx "+++ Fault protection : +++"; FLTSRCx "Fault protection input pin"; FLTSRCx_TXT "<empty>"; FLTDATx "Failt protection safe state :"; CLMODx "+++ Current Limit : +++"; CLSRCx "Current-Limit input pin"; CLSRCx_TXT "<empty>"; CLDATx "Current limit safe state :"; FLTLEBENx "Enable Leading-Edge Blanking to remove glitch on Fault input"; CLLEBENx "Enable Leading-Edge Blanking to remove glitch on Current-Limit input"; LeadEdgeBlkPer_s "Blanking period (s) :"; PHRx "Rising edge of PWM_H trig Leading-Edge Blanking"; PHFx "Falling edge of PWM_H trig Leading-Edge Blanking"; PLRx "Rising edge of PWM_L trig Leading-Edge Blanking"; PLFx "Falling edge of PWM_L trig Leading-Edge Blanking"
      mask help:
      | Multiple instance of this PWM_HS_FEP block might be used within a model to
      |   + set PWM channels with differents characteristics
      |   + update block input at differents time or on specific conditions
      | Model will not compiled if PWM settings of different block violate hardware capabilities.
      |
      | Initial values fields tips (when applicable)
      |   + Scalar input set the same value for all channels enabled.
      |   + Vector  set values for respective channels enabled (first value, first enabled channel...)
      |   + -1 means not used. (for scalar or vector representation)
      mask init:
      | MCHP_PWM_HS_FEP_Callback(gcbh,'INITIALISATION');
      settings: CopyFcn=MCHP_PWM_HS_FEP_Callback(gcbh,'CopyFcn');  PreSaveFcn=MCHP_Fun.PreSaveFcn_DynamicOptions(gcbh);  OpenFcn=MCHP_PWM_HS_FEP_Callback(gcbh,'OPEN');
      mask TypeOptions PWMx_MODSEL: Edge Aligned - Duty Cycle and Phase Shift | Edge Aligned - Rising and Falling Edge | Center Aligned | Center Aligned - Double Update
      mask Callback PWMx_MODSEL: MCHP_PWM_HS_FEP_Callback(gcbh,'UpdateGUI');
      mask TypeOptions PWMx_CLKSEL: Use scaling circuit | Use divider circuit | no scaling
      mask Callback PWMx_CLKSEL: MCHP_PWM_HS_FEP_Callback(gcbh,'UpdateGUI');
      mask TypeOptions PWM_ClockResolution_DIVSEL: Dynamic Options
      mask TypeOptions PWM_ClockResolution_FSCL: Dynamic Options
      mask TypeOptions PWM_ClockResolution_NoScaling: Dynamic Options
      mask TypeOptions PWMx_PMOD: Complementary | Redundant | Push Pull
      mask TypeOptions PWM1_HL: PWMxH & PWMxL output enabled | PWMxH output enabled | PWMxL output enabled | not used | Enabled with NO output
      mask Callback PWM1_HL: MCHP_PWM_HS_FEP_Callback(gcbh,'UpdateGUI');
      mask TypeOptions PWM2_HL: PWMxH & PWMxL output enabled | PWMxH output enabled | PWMxL output enabled | not used | Enabled with NO output
      mask Callback PWM2_HL: MCHP_PWM_HS_FEP_Callback(gcbh,'UpdateGUI');
      mask TypeOptions PWM3_HL: PWMxH & PWMxL output enabled | PWMxH output enabled | PWMxL output enabled | not used | Enabled with NO output
      mask Callback PWM3_HL: MCHP_PWM_HS_FEP_Callback(gcbh,'UpdateGUI');
      mask TypeOptions PWM4_HL: PWMxH & PWMxL output enabled | PWMxH output enabled | PWMxL output enabled | not used | Enabled with NO output
      mask Callback PWM4_HL: MCHP_PWM_HS_FEP_Callback(gcbh,'UpdateGUI');
      mask TypeOptions PWM5_HL: PWMxH & PWMxL output enabled | PWMxH output enabled | PWMxL output enabled | not used | Enabled with NO output
      mask Callback PWM5_HL: MCHP_PWM_HS_FEP_Callback(gcbh,'UpdateGUI');
      mask TypeOptions PWM6_HL: PWMxH & PWMxL output enabled | PWMxH output enabled | PWMxL output enabled | not used | Enabled with NO output
      mask Callback PWM6_HL: MCHP_PWM_HS_FEP_Callback(gcbh,'UpdateGUI');
      mask TypeOptions PWM7_HL: PWMxH & PWMxL output enabled | PWMxH output enabled | PWMxL output enabled | not used | Enabled with NO output
      mask Callback PWM7_HL: MCHP_PWM_HS_FEP_Callback(gcbh,'UpdateGUI');
      mask TypeOptions PWM8_HL: PWMxH & PWMxL output enabled | PWMxH output enabled | PWMxL output enabled | not used | Enabled with NO output
      mask Callback PWM8_HL: MCHP_PWM_HS_FEP_Callback(gcbh,'UpdateGUI');
      mask TypeOptions PWM9_HL: PWMxH & PWMxL output enabled | PWMxH output enabled | PWMxL output enabled | not used | Enabled with NO output
      mask Callback PWM9_HL: MCHP_PWM_HS_FEP_Callback(gcbh,'UpdateGUI');
      mask TypeOptions PWM10_HL: PWMxH & PWMxL output enabled | PWMxH output enabled | PWMxL output enabled | not used | Enabled with NO output
      mask Callback PWM10_HL: MCHP_PWM_HS_FEP_Callback(gcbh,'UpdateGUI');
      mask TypeOptions PWM11_HL: PWMxH & PWMxL output enabled | PWMxH output enabled | PWMxL output enabled | not used | Enabled with NO output
      mask Callback PWM11_HL: MCHP_PWM_HS_FEP_Callback(gcbh,'UpdateGUI');
      mask TypeOptions PWM12_HL: PWMxH & PWMxL output enabled | PWMxH output enabled | PWMxL output enabled | not used | Enabled with NO output
      mask Callback PWM12_HL: MCHP_PWM_HS_FEP_Callback(gcbh,'UpdateGUI');
      mask TypeOptions PWM1_ShowTrig: on | off
      mask Callback PWM1_ShowTrig: MCHP_PWM_HS_FEP_Callback(gcbh,'UpdateGUI');
      mask TypeOptions PWM1_ADTRxEN1: none | ADC Trigger 1 | ADC Trigger 2 | ADC Trigger 1 and ADC Trigger 2
      mask TypeOptions PWM1_ADTRxEN2: none | ADC Trigger 1 | ADC Trigger 2 | ADC Trigger 1 and ADC Trigger 2
      mask TypeOptions PWM1_ADTRxEN3: none | ADC Trigger 1 | ADC Trigger 2 | ADC Trigger 1 and ADC Trigger 2
      mask TypeOptions PWM2_ShowTrig: on | off
      mask Callback PWM2_ShowTrig: MCHP_PWM_HS_FEP_Callback(gcbh,'UpdateGUI');
      mask TypeOptions PWM2_ADTRxEN1: none | ADC Trigger 1 | ADC Trigger 2 | ADC Trigger 1 and ADC Trigger 2
      mask TypeOptions PWM2_ADTRxEN2: none | ADC Trigger 1 | ADC Trigger 2 | ADC Trigger 1 and ADC Trigger 2
      mask TypeOptions PWM2_ADTRxEN3: none | ADC Trigger 1 | ADC Trigger 2 | ADC Trigger 1 and ADC Trigger 2
      mask TypeOptions PWM3_ShowTrig: on | off
      mask Callback PWM3_ShowTrig: MCHP_PWM_HS_FEP_Callback(gcbh,'UpdateGUI');
      mask TypeOptions PWM3_ADTRxEN1: none | ADC Trigger 1 | ADC Trigger 2 | ADC Trigger 1 and ADC Trigger 2
      mask TypeOptions PWM3_ADTRxEN2: none | ADC Trigger 1 | ADC Trigger 2 | ADC Trigger 1 and ADC Trigger 2
      mask TypeOptions PWM3_ADTRxEN3: none | ADC Trigger 1 | ADC Trigger 2 | ADC Trigger 1 and ADC Trigger 2
      mask TypeOptions PWM4_ShowTrig: on | off
      mask Callback PWM4_ShowTrig: MCHP_PWM_HS_FEP_Callback(gcbh,'UpdateGUI');
      mask TypeOptions PWM4_ADTRxEN1: none | ADC Trigger 1 | ADC Trigger 2 | ADC Trigger 1 and ADC Trigger 2
      mask TypeOptions PWM4_ADTRxEN2: none | ADC Trigger 1 | ADC Trigger 2 | ADC Trigger 1 and ADC Trigger 2
      mask TypeOptions PWM4_ADTRxEN3: none | ADC Trigger 1 | ADC Trigger 2 | ADC Trigger 1 and ADC Trigger 2
      mask TypeOptions PWM5_ShowTrig: on | off
      mask Callback PWM5_ShowTrig: MCHP_PWM_HS_FEP_Callback(gcbh,'UpdateGUI');
      mask TypeOptions PWM5_ADTRxEN1: none | ADC Trigger 1 | ADC Trigger 2 | ADC Trigger 1 and ADC Trigger 2
      mask TypeOptions PWM5_ADTRxEN2: none | ADC Trigger 1 | ADC Trigger 2 | ADC Trigger 1 and ADC Trigger 2
      mask TypeOptions PWM5_ADTRxEN3: none | ADC Trigger 1 | ADC Trigger 2 | ADC Trigger 1 and ADC Trigger 2
      mask TypeOptions PWM6_ShowTrig: on | off
      mask Callback PWM6_ShowTrig: MCHP_PWM_HS_FEP_Callback(gcbh,'UpdateGUI');
      mask TypeOptions PWM6_ADTRxEN1: none | ADC Trigger 1 | ADC Trigger 2 | ADC Trigger 1 and ADC Trigger 2
      mask TypeOptions PWM6_ADTRxEN2: none | ADC Trigger 1 | ADC Trigger 2 | ADC Trigger 1 and ADC Trigger 2
      mask TypeOptions PWM6_ADTRxEN3: none | ADC Trigger 1 | ADC Trigger 2 | ADC Trigger 1 and ADC Trigger 2
      mask TypeOptions PWM7_ShowTrig: on | off
      mask Callback PWM7_ShowTrig: MCHP_PWM_HS_FEP_Callback(gcbh,'UpdateGUI');
      mask TypeOptions PWM7_ADTRxEN1: none | ADC Trigger 1 | ADC Trigger 2 | ADC Trigger 1 and ADC Trigger 2
      mask TypeOptions PWM7_ADTRxEN2: none | ADC Trigger 1 | ADC Trigger 2 | ADC Trigger 1 and ADC Trigger 2
      mask TypeOptions PWM7_ADTRxEN3: none | ADC Trigger 1 | ADC Trigger 2 | ADC Trigger 1 and ADC Trigger 2
      mask TypeOptions PWM8_ShowTrig: on | off
      mask Callback PWM8_ShowTrig: MCHP_PWM_HS_FEP_Callback(gcbh,'UpdateGUI');
      mask TypeOptions PWM8_ADTRxEN1: none | ADC Trigger 1 | ADC Trigger 2 | ADC Trigger 1 and ADC Trigger 2
      mask TypeOptions PWM8_ADTRxEN2: none | ADC Trigger 1 | ADC Trigger 2 | ADC Trigger 1 and ADC Trigger 2
      mask TypeOptions PWM8_ADTRxEN3: none | ADC Trigger 1 | ADC Trigger 2 | ADC Trigger 1 and ADC Trigger 2
      mask TypeOptions BlockInput_VectorScalar: Independant Scalar | Vectors (grouped by function)
      mask TypeOptions BlockInput_Period: Not a block input | a Uint raw input (PWMxmax variable represent max period) | a Floating Point input within range [0 1] | a Floating Point input within range [-1 1] | a Floating Point input with physical scaling in (s)
      mask TypeOptions BlockInput_DutyCycle: Not a block input | a Uint raw input (PWMxmax variable represent max period) | a Floating Point input within range [0 1] | a Floating Point input within range [-1 1] | a Floating Point input with physical scaling in (s)
      mask TypeOptions BlockInput_PhaseShift: Not a block input | a Uint raw input (PWMxmax variable represent max period) | a Floating Point input within range [0 1] | a Floating Point input within range [-1 1] | a Floating Point input with physical scaling in (s)
      mask TypeOptions BlockInput_SEVTCMP: Not a block input | a Uint raw input (PWMxmax variable represent max period) | a Floating Point input within range [0 1] | a Floating Point input within range [-1 1] | a Floating Point input with physical scaling in (s)
      mask TypeOptions BlockInput_TRIGx: Not a block input | a Uint raw input (PWMxmax variable represent max period) | a Floating Point input within range [0 1] | a Floating Point input within range [-1 1] | a Floating Point input with physical scaling in (s)
      mask TypeOptions BlockInput_DeadTime: Not a block input | a Uint raw input (PWMxmax variable represent max period) | a Floating Point input within range [0 1] | a Floating Point input within range [-1 1] | a Floating Point input with physical scaling in (s)
      mask TypeOptions DTC: Disabled | Positive dead time (ensure period of time with PWM_H and PWM_L disasserted)
      mask Callback DTC: MCHP_PWM_HS_FEP_Callback(gcbh,'UpdateGUI');
      mask TypeOptions FLTSRC1_DTCMP: Dynamic Options
      mask TypeOptions FLTSRC2_DTCMP: Dynamic Options
      mask TypeOptions FLTSRC3_DTCMP: Dynamic Options
      mask TypeOptions FLTSRC4_DTCMP: Dynamic Options
      mask TypeOptions FLTSRC5_DTCMP: Dynamic Options
      mask TypeOptions FLTSRC6_DTCMP: Dynamic Options
      mask TypeOptions FLTSRC7_DTCMP: Dynamic Options
      mask TypeOptions FLTSRC8_DTCMP: Dynamic Options
      mask TypeOptions FLTSRC9_DTCMP: Dynamic Options
      mask TypeOptions FLTSRC10_DTCMP: Dynamic Options
      mask TypeOptions FLTSRC11_DTCMP: Dynamic Options
      mask TypeOptions FLTSRC12_DTCMP: Dynamic Options
      mask TypeOptions FLTMODx: Disabled | Force PWM output for current cycle. Enable PWM on next cycle | Force PWM output until the FLT block input is 1
      mask Callback FLTMODx: MCHP_PWM_HS_FEP_Callback(gcbh,'UpdateGUI');
      mask TypeOptions FLTSRCx: Dynamic Options
      mask TypeOptions FLTDATx: PWM H/L -> 00 | PWM H/L -> 01 | PWM H/L -> 10 | PWM H/L -> 11 | Not forced
      mask TypeOptions CLMODx: Disabled | Enabled
      mask Callback CLMODx: MCHP_PWM_HS_FEP_Callback(gcbh,'UpdateGUI');
      mask TypeOptions CLSRCx: Dynamic Options
      mask TypeOptions CLDATx: PWM H/L -> 00 | PWM H/L -> 01 | PWM H/L -> 10 | PWM H/L -> 11 | Not forced
      mask Callback FLTLEBENx: MCHP_PWM_HS_FEP_Callback(gcbh,'UpdateGUI');
      mask Callback CLLEBENx: MCHP_PWM_HS_FEP_Callback(gcbh,'UpdateGUI');
      mask Display:
      | fprintf('          PWM HS\n\n          Fine Edge Placement');
      | port_label('input',1,'Duty-Cycle1');
      | port_label('input',2,'Duty-Cycle2');
      | port_label('input',3,'Duty-Cycle3');
